simulink model "Versie2"  (R2019a)
settings: Solver=ode1  StartTime=0.0  StopTime=1.5  FixedStep=Ts_Power  RelTol=1e-3
PostLoadFcn:
  | %% Init for wind PnO models - global system parameters
  | OVERRIDE_SSN_MEMORY_LIMIT=1;
  | Ts=50e-6;
  | % Ts=50e-10;
  | Ts_Power=Ts;
  | Ts_Control=2*Ts;
  | freq = 50;
  | Fnom=freq;
  | Vac=400e3;
InitFcn:
  | %% Init for wind PnO models - global system parameters
  | OVERRIDE_SSN_MEMORY_LIMIT=1;
  | Ts=50e-6;
  | % Ts=50e-10;
  | Ts_Power=Ts;
  | Ts_Control=2*Ts;
  | freq = 50;
  | Fnom=freq;
  | Vac=400e3;
undefined symbols (not defined in the file or in its folder): D11, Delta, den, DiscIntNeverNeededParam, dx, find_system, gcbh, num, out_Buses, out_WindFarms, sps_rtmsupport
libraries: powerlib x258, simulink x112, powerlib_meascontrol x112, eeSinusoidalMeasurement x74, spsVIMeasurementModel x63, elements x52, simulink_extras x44, eePowerMeasurement x26
(part 2 of 27)

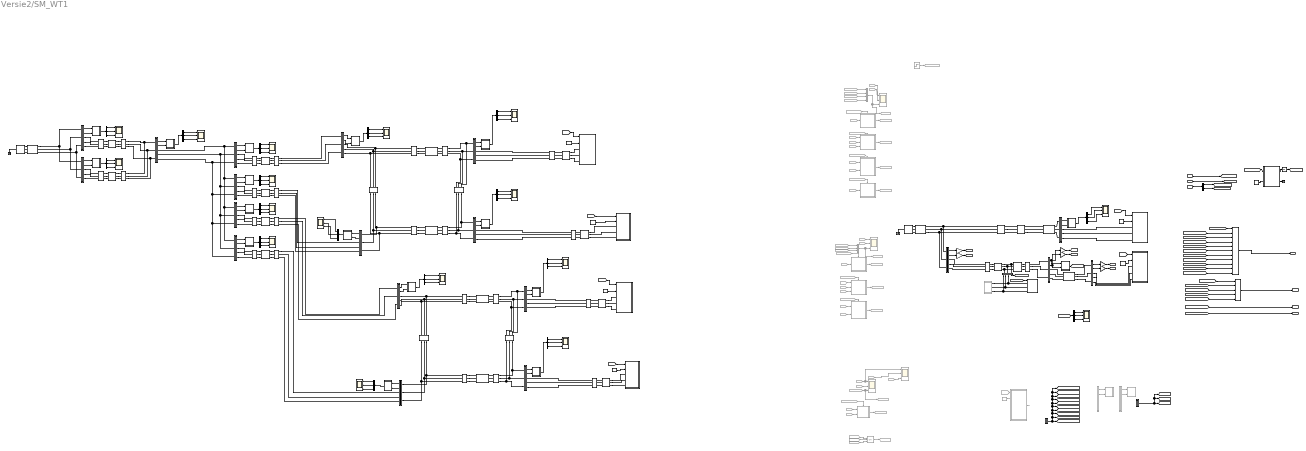
== system Versie2/SM_WT1 ==
  note: Faults
      | with
      | disconnection
      | line
  note: Inputs / Outputs
  note: Analogue Outputs
  note: Digital input (trip signal)
  note: Buses
  note: Wind farms
  note: MODEL TOOLS
  note: Fault
  note: Inputs to this processor core
      | Including blocks to coordinate the communcations
  note: Outputs to monitoring (console)
      | For user interface ('SC_' subsystem)
  note: This subsystem contains the electrical simulation. When performing real-time simulations you cannot view the scopes here. When performing non-real-time simulation (just in matlab/simulink) you can add/view scopes here.
  note: Measurement and protection: bus 2
  note: Measurement and protection: Transformer
  note: Measurement and protection: bus 1
  note: Block protection until model initalised
  wind : Inport
  "FaultParams " : Inport  Port=2
  PlotSelection : Inport  Port=3
   {1..6} (6 alike) : powerlib/Elements/Three-Phase Transformer (Two Windings)  Winding1Connection=Y  Winding2Connection=Yg  CoreType=Three single-phase transformers  SetSaturation=off  Hysteresis=off  DataFile='hysteresis'  SetInitialFlux=off  Measurements=None  UNITS=pu  NominalPower=[1e9 freq]  Winding1=[Vac 0.00083333 0.025]  Winding2=[66e3 0.00083333 0.025]  Rm=500  Lm=Inf  L0=0.5  Saturation=[0 0;0.0024 1.2;1 1.52]  InitialFluxes=[ 0.8 , -0.8 , 0.7 ]  BreakLoop=off  DiscreteSolver=Trapezoidal iterative  DataType=off  TransfoNumber=0
  2500 MVA X0/X1=1 : powerlib/Elements/Three-Phase Mutual Inductance Z1-Z0  LConnTagsString=a|b|c  RConnTagsString=A|B|C  PositiveSequence="[0.1  1.0/(2*pi*freq)] *Vac^2/2500e6/10"  ZeroSequence="[0.3  3.0/(2*pi*freq)] *Vac^2/2500e6/10"
      settings: SourceProductBaseCode=PS
  2500 MVA X0/X1=2 : powerlib/Elements/Three-Phase Mutual Inductance Z1-Z0  LConnTagsString=a|b|c  RConnTagsString=A|B|C  PositiveSequence="[0.1  1.0/(2*pi*freq)] *Vac^2/2500e6/10"  ZeroSequence="[0.3  3.0/(2*pi*freq)] *Vac^2/2500e6/10"
      settings: SourceProductBaseCode=PS
  5 km fault1 : powerlib/Elements/Three-Phase PI Section Line  LConnTagsString=a|b|c  RConnTagsString=A|B|C  Frequency=freq  Resistances=[0.1153 0.413]  Inductances=[1.05e-3 3.32e-3]  Capacitances=[11.33e-009 5.01e-009]  Length=20
  5 km fault2 : powerlib/Elements/Three-Phase PI Section Line  LConnTagsString=a|b|c  RConnTagsString=A|B|C  Frequency=freq  Resistances=[0.1153 0.413]  Inductances=[1.05e-3 3.32e-3]  Capacitances=[11.33e-009 5.01e-009]  Length=20
  5 km series1 : powerlib/Elements/Three-Phase PI Section Line  LConnTagsString=a|b|c  RConnTagsString=A|B|C  Frequency=freq  Resistances=[0.1153 0.413]  Inductances=[1.05e-3 3.32e-3]  Capacitances=[11.33e-009 5.01e-009]  Length=20
  5 km series{3..8,11,17,28,34} (10 alike) : powerlib/Elements/Three-Phase PI Section Line  LConnTagsString=a|b|c  RConnTagsString=A|B|C  Frequency=freq  Resistances=[0.1153 0.413]  Inductances=[1.05e-3 3.32e-3]  Capacitances=[11.33e-009 5.01e-009]  Length=10
  5 km series2 : powerlib/Elements/Three-Phase PI Section Line  LConnTagsString=a|b|c  RConnTagsString=A|B|C  Frequency=freq  Resistances=[0.1153 0.413]  Inductances=[1.05e-3 3.32e-3]  Capacitances=[11.33e-009 5.01e-009]  Length=20
  Bus Creator : BusCreator  Commented=on  Inputs=4
  Bus Creator1 : BusCreator  Commented=on  Inputs=3
  Bus Selector : BusSelector  OutputSignals=Turbine,Bus
  Bus Selector{1..17} (17 alike) : BusSelector  OutputSignals=Vabc,Iabc,PQ
  BusA : Subsystem  DialogController=POWERSYS.PowerSysDialog  LoadFcn=sps_rtmsupport('LoadFcn',gcbh);  StartFcn=sps_rtmsupport('StartFcn',gcbh);  StopFcn=sps_rtmsupport('StopFcn',gcbh);  mask(Three-Phase VI Measurement){VoltageMeasurement=phase-to-ground, SetLabelV=off, LabelV=Vabc, Vpu=off, VpuLL=off, CurrentMeasurement=yes, SetLabelI=off, LabelI=Iabc, Ipu=off, Pbase=100e6, Vbase=500e3, OutputType=Complex, PhasorSimulation=off, PSBequivalent=0}
      mask prompts: VoltageMeasurement "Voltage measurement"; SetLabelV "Use a label"; LabelV "Signal label  (use a From block to collect this signal)"; Vpu "Voltages in pu,  based on peak value of nominal phase-to-ground voltage"; VpuLL "Voltages in pu,  based on peak value of nominal phase-to-phase  voltage"; CurrentMeasurement "Current measurement"; SetLabelI "Use a label"; LabelI "Signal label  (use a From block to collect this signal)"; Ipu "Currents in pu"; Pbase "Base power ( VA 3 phase)"; Vbase "Nominal voltage used for pu measurement (Vrms phase-phase) :"; OutputType "Output signals in:"; PhasorSimulation "Phasor simulation (internal use)"; PSBequivalent "Equivalent circuit (internal use)"
      mask help:
      | Ideal three-phase voltage and current measurements.
      |
      | The block can output the voltages and currents in per unit values or in volts and amperes.
      mask init:
      | block = gcb;
      | Kv=1;
      | Ki=1;
      | [Kv,Ki] = powericon('ThreePhaseVIMeasurementParam',block,Vpu,VpuLL,Ipu,Vbase,Pbase,PhasorSimulation,OutputType);
      | powericon('ThreePhaseVIMeasurementCback',block);
      | power_initmask();
      settings: CopyFcn=sps_rtmsupport('CopyFcn',gcbh); powericon('ThreePhaseVIMeasurementCopy',gcb)  DeleteFcn=sps_rtmsupport('DeleteFcn',gcbh);  UndoDeleteFcn=sps_rtmsupport('UndoDeleteFcn',gcbh);  ModelCloseFcn=sps_rtmsupport('ModelCloseFcn',gcbh);  PreSaveFcn="sps_rtmsupport('PreSaveFcn',gcbh);  set_param(gcb,'LinkStatus','restore')"  PostSaveFcn=sps_rtmsupport('PostSaveFcn',gcbh);  NameChangeFcn=sps_rtmsupport('NameChangeFcn',gcbh);  PreCopyFcn=sps_rtmsupport('PreCopyFcn',gcbh);  OpenFcn=sps_rtmsupport('OpenFcn',gcbh, [1 2 4 5 6 7 9 -12 13]);  CloseFcn=sps_rtmsupport('CloseFcn',gcbh);  PreDeleteFcn=sps_rtmsupport('PreDeleteFcn',gcbh);
      mask Help: helpview(psbhelp)
      mask TypeOptions VoltageMeasurement: no | phase-to-ground | phase-to-phase
      mask Callback VoltageMeasurement: powericon('ThreePhaseVIMeasurementCback',gcb,'Vselector');
      mask Callback SetLabelV: powericon('ThreePhaseVIMeasurementCback',gcb,'');
      mask Callback Vpu: powericon('ThreePhaseVIMeasurementCback',gcb,'Vpu');
      mask Callback VpuLL: powericon('ThreePhaseVIMeasurementCback',gcb,'VpuLL');
      mask TypeOptions CurrentMeasurement: no | yes
      mask Callback CurrentMeasurement: powericon('ThreePhaseVIMeasurementCback',gcb,'');
      mask Callback SetLabelI: powericon('ThreePhaseVIMeasurementCback',gcb,'');
      mask Callback LabelI: powericon('ThreePhaseVIMeasurementCback',gcb,'');
      mask Callback Ipu: powericon('ThreePhaseVIMeasurementCback',gcb,'');
      mask TypeOptions OutputType: Complex | Real-Imag | Magnitude-Angle | Magnitude
  BusB : Subsystem  Commented=on  DialogController=POWERSYS.PowerSysDialog  LoadFcn=sps_rtmsupport('LoadFcn',gcbh);  StartFcn=sps_rtmsupport('StartFcn',gcbh);  StopFcn=sps_rtmsupport('StopFcn',gcbh);  mask(Three-Phase VI Measurement){VoltageMeasurement=phase-to-ground, SetLabelV=off, LabelV=Vabc, Vpu=off, VpuLL=off, CurrentMeasurement=yes, SetLabelI=off, LabelI=Iabc, Ipu=off, Pbase=100e6, Vbase=500e3, OutputType=Complex, PhasorSimulation=off, PSBequivalent=0}
      mask prompts: VoltageMeasurement "Voltage measurement"; SetLabelV "Use a label"; LabelV "Signal label  (use a From block to collect this signal)"; Vpu "Voltages in pu,  based on peak value of nominal phase-to-ground voltage"; VpuLL "Voltages in pu,  based on peak value of nominal phase-to-phase  voltage"; CurrentMeasurement "Current measurement"; SetLabelI "Use a label"; LabelI "Signal label  (use a From block to collect this signal)"; Ipu "Currents in pu"; Pbase "Base power ( VA 3 phase)"; Vbase "Nominal voltage used for pu measurement (Vrms phase-phase) :"; OutputType "Output signals in:"; PhasorSimulation "Phasor simulation (internal use)"; PSBequivalent "Equivalent circuit (internal use)"
      mask help:
      | Ideal three-phase voltage and current measurements.
      |
      | The block can output the voltages and currents in per unit values or in volts and amperes.
      mask init: same as Versie2/SM_WT1/BusA
      settings: CopyFcn=sps_rtmsupport('CopyFcn',gcbh); powericon('ThreePhaseVIMeasurementCopy',gcb)  DeleteFcn=sps_rtmsupport('DeleteFcn',gcbh);  UndoDeleteFcn=sps_rtmsupport('UndoDeleteFcn',gcbh);  ModelCloseFcn=sps_rtmsupport('ModelCloseFcn',gcbh);  PreSaveFcn="sps_rtmsupport('PreSaveFcn',gcbh);  set_param(gcb,'LinkStatus','restore')"  PostSaveFcn=sps_rtmsupport('PostSaveFcn',gcbh);  NameChangeFcn=sps_rtmsupport('NameChangeFcn',gcbh);  PreCopyFcn=sps_rtmsupport('PreCopyFcn',gcbh);  OpenFcn=sps_rtmsupport('OpenFcn',gcbh, [1 2 4 5 6 7 9 -12 13]);  CloseFcn=sps_rtmsupport('CloseFcn',gcbh);  PreDeleteFcn=sps_rtmsupport('PreDeleteFcn',gcbh);
      mask Help: helpview(psbhelp)
      mask TypeOptions VoltageMeasurement: no | phase-to-ground | phase-to-phase
      mask Callback VoltageMeasurement: powericon('ThreePhaseVIMeasurementCback',gcb,'Vselector');
      mask Callback SetLabelV: powericon('ThreePhaseVIMeasurementCback',gcb,'');
      mask Callback Vpu: powericon('ThreePhaseVIMeasurementCback',gcb,'Vpu');
      mask Callback VpuLL: powericon('ThreePhaseVIMeasurementCback',gcb,'VpuLL');
      mask TypeOptions CurrentMeasurement: no | yes
      mask Callback CurrentMeasurement: powericon('ThreePhaseVIMeasurementCback',gcb,'');
      mask Callback SetLabelI: powericon('ThreePhaseVIMeasurementCback',gcb,'');
      mask Callback LabelI: powericon('ThreePhaseVIMeasurementCback',gcb,'');
      mask Callback Ipu: powericon('ThreePhaseVIMeasurementCback',gcb,'');
      mask TypeOptions OutputType: Complex | Real-Imag | Magnitude-Angle | Magnitude
  BusC : Subsystem  DialogController=POWERSYS.PowerSysDialog  LoadFcn=sps_rtmsupport('LoadFcn',gcbh);  StartFcn=sps_rtmsupport('StartFcn',gcbh);  StopFcn=sps_rtmsupport('StopFcn',gcbh);  mask(Three-Phase VI Measurement){VoltageMeasurement=phase-to-ground, SetLabelV=off, LabelV=Vabc, Vpu=off, VpuLL=off, CurrentMeasurement=yes, SetLabelI=off, LabelI=Iabc, Ipu=off, Pbase=100e6, Vbase=500e3, OutputType=Complex, PhasorSimulation=off, PSBequivalent=0}
      mask prompts: VoltageMeasurement "Voltage measurement"; SetLabelV "Use a label"; LabelV "Signal label  (use a From block to collect this signal)"; Vpu "Voltages in pu,  based on peak value of nominal phase-to-ground voltage"; VpuLL "Voltages in pu,  based on peak value of nominal phase-to-phase  voltage"; CurrentMeasurement "Current measurement"; SetLabelI "Use a label"; LabelI "Signal label  (use a From block to collect this signal)"; Ipu "Currents in pu"; Pbase "Base power ( VA 3 phase)"; Vbase "Nominal voltage used for pu measurement (Vrms phase-phase) :"; OutputType "Output signals in:"; PhasorSimulation "Phasor simulation (internal use)"; PSBequivalent "Equivalent circuit (internal use)"
      mask help:
      | Ideal three-phase voltage and current measurements.
      |
      | The block can output the voltages and currents in per unit values or in volts and amperes.
      mask init: same as Versie2/SM_WT1/BusA
      settings: CopyFcn=sps_rtmsupport('CopyFcn',gcbh); powericon('ThreePhaseVIMeasurementCopy',gcb)  DeleteFcn=sps_rtmsupport('DeleteFcn',gcbh);  UndoDeleteFcn=sps_rtmsupport('UndoDeleteFcn',gcbh);  ModelCloseFcn=sps_rtmsupport('ModelCloseFcn',gcbh);  PreSaveFcn="sps_rtmsupport('PreSaveFcn',gcbh);  set_param(gcb,'LinkStatus','restore')"  PostSaveFcn=sps_rtmsupport('PostSaveFcn',gcbh);  NameChangeFcn=sps_rtmsupport('NameChangeFcn',gcbh);  PreCopyFcn=sps_rtmsupport('PreCopyFcn',gcbh);  OpenFcn=sps_rtmsupport('OpenFcn',gcbh, [1 2 4 5 6 7 9 -12 13]);  CloseFcn=sps_rtmsupport('CloseFcn',gcbh);  PreDeleteFcn=sps_rtmsupport('PreDeleteFcn',gcbh);
      mask Help: helpview(psbhelp)
      mask TypeOptions VoltageMeasurement: no | phase-to-ground | phase-to-phase
      mask Callback VoltageMeasurement: powericon('ThreePhaseVIMeasurementCback',gcb,'Vselector');
      mask Callback SetLabelV: powericon('ThreePhaseVIMeasurementCback',gcb,'');
      mask Callback Vpu: powericon('ThreePhaseVIMeasurementCback',gcb,'Vpu');
      mask Callback VpuLL: powericon('ThreePhaseVIMeasurementCback',gcb,'VpuLL');
      mask TypeOptions CurrentMeasurement: no | yes
      mask Callback CurrentMeasurement: powericon('ThreePhaseVIMeasurementCback',gcb,'');
      mask Callback SetLabelI: powericon('ThreePhaseVIMeasurementCback',gcb,'');
      mask Callback LabelI: powericon('ThreePhaseVIMeasurementCback',gcb,'');
      mask Callback Ipu: powericon('ThreePhaseVIMeasurementCback',gcb,'');
      mask TypeOptions OutputType: Complex | Real-Imag | Magnitude-Angle | Magnitude
  BusC1 : Subsystem  DialogController=POWERSYS.PowerSysDialog  LoadFcn=sps_rtmsupport('LoadFcn',gcbh);  StartFcn=sps_rtmsupport('StartFcn',gcbh);  StopFcn=sps_rtmsupport('StopFcn',gcbh);  mask(Three-Phase VI Measurement){VoltageMeasurement=phase-to-ground, SetLabelV=off, LabelV=Vabc, Vpu=off, VpuLL=off, CurrentMeasurement=yes, SetLabelI=off, LabelI=Iabc, Ipu=off, Pbase=100e6, Vbase=500e3, OutputType=Complex, PhasorSimulation=off, PSBequivalent=0}
      mask prompts: VoltageMeasurement "Voltage measurement"; SetLabelV "Use a label"; LabelV "Signal label  (use a From block to collect this signal)"; Vpu "Voltages in pu,  based on peak value of nominal phase-to-ground voltage"; VpuLL "Voltages in pu,  based on peak value of nominal phase-to-phase  voltage"; CurrentMeasurement "Current measurement"; SetLabelI "Use a label"; LabelI "Signal label  (use a From block to collect this signal)"; Ipu "Currents in pu"; Pbase "Base power ( VA 3 phase)"; Vbase "Nominal voltage used for pu measurement (Vrms phase-phase) :"; OutputType "Output signals in:"; PhasorSimulation "Phasor simulation (internal use)"; PSBequivalent "Equivalent circuit (internal use)"
      mask help:
      | Ideal three-phase voltage and current measurements.
      |
      | The block can output the voltages and currents in per unit values or in volts and amperes.
      mask init: same as Versie2/SM_WT1/BusA
      settings: CopyFcn=sps_rtmsupport('CopyFcn',gcbh); powericon('ThreePhaseVIMeasurementCopy',gcb)  DeleteFcn=sps_rtmsupport('DeleteFcn',gcbh);  UndoDeleteFcn=sps_rtmsupport('UndoDeleteFcn',gcbh);  ModelCloseFcn=sps_rtmsupport('ModelCloseFcn',gcbh);  PreSaveFcn="sps_rtmsupport('PreSaveFcn',gcbh);  set_param(gcb,'LinkStatus','restore')"  PostSaveFcn=sps_rtmsupport('PostSaveFcn',gcbh);  NameChangeFcn=sps_rtmsupport('NameChangeFcn',gcbh);  PreCopyFcn=sps_rtmsupport('PreCopyFcn',gcbh);  OpenFcn=sps_rtmsupport('OpenFcn',gcbh, [1 2 4 5 6 7 9 -12 13]);  CloseFcn=sps_rtmsupport('CloseFcn',gcbh);  PreDeleteFcn=sps_rtmsupport('PreDeleteFcn',gcbh);
      mask Help: helpview(psbhelp)
      mask TypeOptions VoltageMeasurement: no | phase-to-ground | phase-to-phase
      mask Callback VoltageMeasurement: powericon('ThreePhaseVIMeasurementCback',gcb,'Vselector');
      mask Callback SetLabelV: powericon('ThreePhaseVIMeasurementCback',gcb,'');
      mask Callback Vpu: powericon('ThreePhaseVIMeasurementCback',gcb,'Vpu');
      mask Callback VpuLL: powericon('ThreePhaseVIMeasurementCback',gcb,'VpuLL');
      mask TypeOptions CurrentMeasurement: no | yes
      mask Callback CurrentMeasurement: powericon('ThreePhaseVIMeasurementCback',gcb,'');
      mask Callback SetLabelI: powericon('ThreePhaseVIMeasurementCback',gcb,'');
      mask Callback LabelI: powericon('ThreePhaseVIMeasurementCback',gcb,'');
      mask Callback Ipu: powericon('ThreePhaseVIMeasurementCback',gcb,'');
      mask TypeOptions OutputType: Complex | Real-Imag | Magnitude-Angle | Magnitude
  BusC10 : Subsystem  DialogController=POWERSYS.PowerSysDialog  LoadFcn=sps_rtmsupport('LoadFcn',gcbh);  StartFcn=sps_rtmsupport('StartFcn',gcbh);  StopFcn=sps_rtmsupport('StopFcn',gcbh);  mask(Three-Phase VI Measurement){VoltageMeasurement=phase-to-ground, SetLabelV=off, LabelV=Vabc, Vpu=off, VpuLL=off, CurrentMeasurement=yes, SetLabelI=off, LabelI=Iabc, Ipu=off, Pbase=100e6, Vbase=500e3, OutputType=Complex, PhasorSimulation=off, PSBequivalent=0}
      mask prompts: VoltageMeasurement "Voltage measurement"; SetLabelV "Use a label"; LabelV "Signal label  (use a From block to collect this signal)"; Vpu "Voltages in pu,  based on peak value of nominal phase-to-ground voltage"; VpuLL "Voltages in pu,  based on peak value of nominal phase-to-phase  voltage"; CurrentMeasurement "Current measurement"; SetLabelI "Use a label"; LabelI "Signal label  (use a From block to collect this signal)"; Ipu "Currents in pu"; Pbase "Base power ( VA 3 phase)"; Vbase "Nominal voltage used for pu measurement (Vrms phase-phase) :"; OutputType "Output signals in:"; PhasorSimulation "Phasor simulation (internal use)"; PSBequivalent "Equivalent circuit (internal use)"
      mask help:
      | Ideal three-phase voltage and current measurements.
      |
      | The block can output the voltages and currents in per unit values or in volts and amperes.
      mask init: same as Versie2/SM_WT1/BusA
      settings: CopyFcn=sps_rtmsupport('CopyFcn',gcbh); powericon('ThreePhaseVIMeasurementCopy',gcb)  DeleteFcn=sps_rtmsupport('DeleteFcn',gcbh);  UndoDeleteFcn=sps_rtmsupport('UndoDeleteFcn',gcbh);  ModelCloseFcn=sps_rtmsupport('ModelCloseFcn',gcbh);  PreSaveFcn="sps_rtmsupport('PreSaveFcn',gcbh);  set_param(gcb,'LinkStatus','restore')"  PostSaveFcn=sps_rtmsupport('PostSaveFcn',gcbh);  NameChangeFcn=sps_rtmsupport('NameChangeFcn',gcbh);  PreCopyFcn=sps_rtmsupport('PreCopyFcn',gcbh);  OpenFcn=sps_rtmsupport('OpenFcn',gcbh, [1 2 4 5 6 7 9 -12 13]);  CloseFcn=sps_rtmsupport('CloseFcn',gcbh);  PreDeleteFcn=sps_rtmsupport('PreDeleteFcn',gcbh);
      mask Help: helpview(psbhelp)
      mask TypeOptions VoltageMeasurement: no | phase-to-ground | phase-to-phase
      mask Callback VoltageMeasurement: powericon('ThreePhaseVIMeasurementCback',gcb,'Vselector');
      mask Callback SetLabelV: powericon('ThreePhaseVIMeasurementCback',gcb,'');
      mask Callback Vpu: powericon('ThreePhaseVIMeasurementCback',gcb,'Vpu');
      mask Callback VpuLL: powericon('ThreePhaseVIMeasurementCback',gcb,'VpuLL');
      mask TypeOptions CurrentMeasurement: no | yes
      mask Callback CurrentMeasurement: powericon('ThreePhaseVIMeasurementCback',gcb,'');
      mask Callback SetLabelI: powericon('ThreePhaseVIMeasurementCback',gcb,'');
      mask Callback LabelI: powericon('ThreePhaseVIMeasurementCback',gcb,'');
      mask Callback Ipu: powericon('ThreePhaseVIMeasurementCback',gcb,'');
      mask TypeOptions OutputType: Complex | Real-Imag | Magnitude-Angle | Magnitude
  BusC11 : Subsystem  DialogController=POWERSYS.PowerSysDialog  LoadFcn=sps_rtmsupport('LoadFcn',gcbh);  StartFcn=sps_rtmsupport('StartFcn',gcbh);  StopFcn=sps_rtmsupport('StopFcn',gcbh);  mask(Three-Phase VI Measurement){VoltageMeasurement=phase-to-ground, SetLabelV=off, LabelV=Vabc, Vpu=off, VpuLL=off, CurrentMeasurement=yes, SetLabelI=off, LabelI=Iabc, Ipu=off, Pbase=100e6, Vbase=500e3, OutputType=Complex, PhasorSimulation=off, PSBequivalent=0}
      mask prompts: VoltageMeasurement "Voltage measurement"; SetLabelV "Use a label"; LabelV "Signal label  (use a From block to collect this signal)"; Vpu "Voltages in pu,  based on peak value of nominal phase-to-ground voltage"; VpuLL "Voltages in pu,  based on peak value of nominal phase-to-phase  voltage"; CurrentMeasurement "Current measurement"; SetLabelI "Use a label"; LabelI "Signal label  (use a From block to collect this signal)"; Ipu "Currents in pu"; Pbase "Base power ( VA 3 phase)"; Vbase "Nominal voltage used for pu measurement (Vrms phase-phase) :"; OutputType "Output signals in:"; PhasorSimulation "Phasor simulation (internal use)"; PSBequivalent "Equivalent circuit (internal use)"
      mask help:
      | Ideal three-phase voltage and current measurements.
      |
      | The block can output the voltages and currents in per unit values or in volts and amperes.
      mask init: same as Versie2/SM_WT1/BusA
      settings: CopyFcn=sps_rtmsupport('CopyFcn',gcbh); powericon('ThreePhaseVIMeasurementCopy',gcb)  DeleteFcn=sps_rtmsupport('DeleteFcn',gcbh);  UndoDeleteFcn=sps_rtmsupport('UndoDeleteFcn',gcbh);  ModelCloseFcn=sps_rtmsupport('ModelCloseFcn',gcbh);  PreSaveFcn="sps_rtmsupport('PreSaveFcn',gcbh);  set_param(gcb,'LinkStatus','restore')"  PostSaveFcn=sps_rtmsupport('PostSaveFcn',gcbh);  NameChangeFcn=sps_rtmsupport('NameChangeFcn',gcbh);  PreCopyFcn=sps_rtmsupport('PreCopyFcn',gcbh);  OpenFcn=sps_rtmsupport('OpenFcn',gcbh, [1 2 4 5 6 7 9 -12 13]);  CloseFcn=sps_rtmsupport('CloseFcn',gcbh);  PreDeleteFcn=sps_rtmsupport('PreDeleteFcn',gcbh);
      mask Help: helpview(psbhelp)
      mask TypeOptions VoltageMeasurement: no | phase-to-ground | phase-to-phase
      mask Callback VoltageMeasurement: powericon('ThreePhaseVIMeasurementCback',gcb,'Vselector');
      mask Callback SetLabelV: powericon('ThreePhaseVIMeasurementCback',gcb,'');
      mask Callback Vpu: powericon('ThreePhaseVIMeasurementCback',gcb,'Vpu');
      mask Callback VpuLL: powericon('ThreePhaseVIMeasurementCback',gcb,'VpuLL');
      mask TypeOptions CurrentMeasurement: no | yes
      mask Callback CurrentMeasurement: powericon('ThreePhaseVIMeasurementCback',gcb,'');
      mask Callback SetLabelI: powericon('ThreePhaseVIMeasurementCback',gcb,'');
      mask Callback LabelI: powericon('ThreePhaseVIMeasurementCback',gcb,'');
      mask Callback Ipu: powericon('ThreePhaseVIMeasurementCback',gcb,'');
      mask TypeOptions OutputType: Complex | Real-Imag | Magnitude-Angle | Magnitude
  BusC12 : Subsystem  DialogController=POWERSYS.PowerSysDialog  LoadFcn=sps_rtmsupport('LoadFcn',gcbh);  StartFcn=sps_rtmsupport('StartFcn',gcbh);  StopFcn=sps_rtmsupport('StopFcn',gcbh);  mask(Three-Phase VI Measurement){VoltageMeasurement=phase-to-ground, SetLabelV=off, LabelV=Vabc, Vpu=off, VpuLL=off, CurrentMeasurement=yes, SetLabelI=off, LabelI=Iabc, Ipu=off, Pbase=100e6, Vbase=500e3, OutputType=Complex, PhasorSimulation=off, PSBequivalent=0}
      mask prompts: VoltageMeasurement "Voltage measurement"; SetLabelV "Use a label"; LabelV "Signal label  (use a From block to collect this signal)"; Vpu "Voltages in pu,  based on peak value of nominal phase-to-ground voltage"; VpuLL "Voltages in pu,  based on peak value of nominal phase-to-phase  voltage"; CurrentMeasurement "Current measurement"; SetLabelI "Use a label"; LabelI "Signal label  (use a From block to collect this signal)"; Ipu "Currents in pu"; Pbase "Base power ( VA 3 phase)"; Vbase "Nominal voltage used for pu measurement (Vrms phase-phase) :"; OutputType "Output signals in:"; PhasorSimulation "Phasor simulation (internal use)"; PSBequivalent "Equivalent circuit (internal use)"
      mask help:
      | Ideal three-phase voltage and current measurements.
      |
      | The block can output the voltages and currents in per unit values or in volts and amperes.
      mask init: same as Versie2/SM_WT1/BusA
      settings: CopyFcn=sps_rtmsupport('CopyFcn',gcbh); powericon('ThreePhaseVIMeasurementCopy',gcb)  DeleteFcn=sps_rtmsupport('DeleteFcn',gcbh);  UndoDeleteFcn=sps_rtmsupport('UndoDeleteFcn',gcbh);  ModelCloseFcn=sps_rtmsupport('ModelCloseFcn',gcbh);  PreSaveFcn="sps_rtmsupport('PreSaveFcn',gcbh);  set_param(gcb,'LinkStatus','restore')"  PostSaveFcn=sps_rtmsupport('PostSaveFcn',gcbh);  NameChangeFcn=sps_rtmsupport('NameChangeFcn',gcbh);  PreCopyFcn=sps_rtmsupport('PreCopyFcn',gcbh);  OpenFcn=sps_rtmsupport('OpenFcn',gcbh, [1 2 4 5 6 7 9 -12 13]);  CloseFcn=sps_rtmsupport('CloseFcn',gcbh);  PreDeleteFcn=sps_rtmsupport('PreDeleteFcn',gcbh);
      mask Help: helpview(psbhelp)
      mask TypeOptions VoltageMeasurement: no | phase-to-ground | phase-to-phase
      mask Callback VoltageMeasurement: powericon('ThreePhaseVIMeasurementCback',gcb,'Vselector');
      mask Callback SetLabelV: powericon('ThreePhaseVIMeasurementCback',gcb,'');
      mask Callback Vpu: powericon('ThreePhaseVIMeasurementCback',gcb,'Vpu');
      mask Callback VpuLL: powericon('ThreePhaseVIMeasurementCback',gcb,'VpuLL');
      mask TypeOptions CurrentMeasurement: no | yes
      mask Callback CurrentMeasurement: powericon('ThreePhaseVIMeasurementCback',gcb,'');
      mask Callback SetLabelI: powericon('ThreePhaseVIMeasurementCback',gcb,'');
      mask Callback LabelI: powericon('ThreePhaseVIMeasurementCback',gcb,'');
      mask Callback Ipu: powericon('ThreePhaseVIMeasurementCback',gcb,'');
      mask TypeOptions OutputType: Complex | Real-Imag | Magnitude-Angle | Magnitude
  BusC13 : Subsystem  DialogController=POWERSYS.PowerSysDialog  LoadFcn=sps_rtmsupport('LoadFcn',gcbh);  StartFcn=sps_rtmsupport('StartFcn',gcbh);  StopFcn=sps_rtmsupport('StopFcn',gcbh);  mask(Three-Phase VI Measurement){VoltageMeasurement=phase-to-ground, SetLabelV=off, LabelV=Vabc, Vpu=off, VpuLL=off, CurrentMeasurement=yes, SetLabelI=off, LabelI=Iabc, Ipu=off, Pbase=100e6, Vbase=500e3, OutputType=Complex, PhasorSimulation=off, PSBequivalent=0}
      mask prompts: VoltageMeasurement "Voltage measurement"; SetLabelV "Use a label"; LabelV "Signal label  (use a From block to collect this signal)"; Vpu "Voltages in pu,  based on peak value of nominal phase-to-ground voltage"; VpuLL "Voltages in pu,  based on peak value of nominal phase-to-phase  voltage"; CurrentMeasurement "Current measurement"; SetLabelI "Use a label"; LabelI "Signal label  (use a From block to collect this signal)"; Ipu "Currents in pu"; Pbase "Base power ( VA 3 phase)"; Vbase "Nominal voltage used for pu measurement (Vrms phase-phase) :"; OutputType "Output signals in:"; PhasorSimulation "Phasor simulation (internal use)"; PSBequivalent "Equivalent circuit (internal use)"
      mask help:
      | Ideal three-phase voltage and current measurements.
      |
      | The block can output the voltages and currents in per unit values or in volts and amperes.
      mask init: same as Versie2/SM_WT1/BusA
      settings: CopyFcn=sps_rtmsupport('CopyFcn',gcbh); powericon('ThreePhaseVIMeasurementCopy',gcb)  DeleteFcn=sps_rtmsupport('DeleteFcn',gcbh);  UndoDeleteFcn=sps_rtmsupport('UndoDeleteFcn',gcbh);  ModelCloseFcn=sps_rtmsupport('ModelCloseFcn',gcbh);  PreSaveFcn="sps_rtmsupport('PreSaveFcn',gcbh);  set_param(gcb,'LinkStatus','restore')"  PostSaveFcn=sps_rtmsupport('PostSaveFcn',gcbh);  NameChangeFcn=sps_rtmsupport('NameChangeFcn',gcbh);  PreCopyFcn=sps_rtmsupport('PreCopyFcn',gcbh);  OpenFcn=sps_rtmsupport('OpenFcn',gcbh, [1 2 4 5 6 7 9 -12 13]);  CloseFcn=sps_rtmsupport('CloseFcn',gcbh);  PreDeleteFcn=sps_rtmsupport('PreDeleteFcn',gcbh);
      mask Help: helpview(psbhelp)
      mask TypeOptions VoltageMeasurement: no | phase-to-ground | phase-to-phase
      mask Callback VoltageMeasurement: powericon('ThreePhaseVIMeasurementCback',gcb,'Vselector');
      mask Callback SetLabelV: powericon('ThreePhaseVIMeasurementCback',gcb,'');
      mask Callback Vpu: powericon('ThreePhaseVIMeasurementCback',gcb,'Vpu');
      mask Callback VpuLL: powericon('ThreePhaseVIMeasurementCback',gcb,'VpuLL');
      mask TypeOptions CurrentMeasurement: no | yes
      mask Callback CurrentMeasurement: powericon('ThreePhaseVIMeasurementCback',gcb,'');
      mask Callback SetLabelI: powericon('ThreePhaseVIMeasurementCback',gcb,'');
      mask Callback LabelI: powericon('ThreePhaseVIMeasurementCback',gcb,'');
      mask Callback Ipu: powericon('ThreePhaseVIMeasurementCback',gcb,'');
      mask TypeOptions OutputType: Complex | Real-Imag | Magnitude-Angle | Magnitude
  BusC14 : Subsystem  DialogController=POWERSYS.PowerSysDialog  LoadFcn=sps_rtmsupport('LoadFcn',gcbh);  StartFcn=sps_rtmsupport('StartFcn',gcbh);  StopFcn=sps_rtmsupport('StopFcn',gcbh);  mask(Three-Phase VI Measurement){VoltageMeasurement=phase-to-ground, SetLabelV=off, LabelV=Vabc, Vpu=off, VpuLL=off, CurrentMeasurement=yes, SetLabelI=off, LabelI=Iabc, Ipu=off, Pbase=100e6, Vbase=500e3, OutputType=Complex, PhasorSimulation=off, PSBequivalent=0}
      mask prompts: VoltageMeasurement "Voltage measurement"; SetLabelV "Use a label"; LabelV "Signal label  (use a From block to collect this signal)"; Vpu "Voltages in pu,  based on peak value of nominal phase-to-ground voltage"; VpuLL "Voltages in pu,  based on peak value of nominal phase-to-phase  voltage"; CurrentMeasurement "Current measurement"; SetLabelI "Use a label"; LabelI "Signal label  (use a From block to collect this signal)"; Ipu "Currents in pu"; Pbase "Base power ( VA 3 phase)"; Vbase "Nominal voltage used for pu measurement (Vrms phase-phase) :"; OutputType "Output signals in:"; PhasorSimulation "Phasor simulation (internal use)"; PSBequivalent "Equivalent circuit (internal use)"
      mask help:
      | Ideal three-phase voltage and current measurements.
      |
      | The block can output the voltages and currents in per unit values or in volts and amperes.
      mask init: same as Versie2/SM_WT1/BusA
      settings: CopyFcn=sps_rtmsupport('CopyFcn',gcbh); powericon('ThreePhaseVIMeasurementCopy',gcb)  DeleteFcn=sps_rtmsupport('DeleteFcn',gcbh);  UndoDeleteFcn=sps_rtmsupport('UndoDeleteFcn',gcbh);  ModelCloseFcn=sps_rtmsupport('ModelCloseFcn',gcbh);  PreSaveFcn="sps_rtmsupport('PreSaveFcn',gcbh);  set_param(gcb,'LinkStatus','restore')"  PostSaveFcn=sps_rtmsupport('PostSaveFcn',gcbh);  NameChangeFcn=sps_rtmsupport('NameChangeFcn',gcbh);  PreCopyFcn=sps_rtmsupport('PreCopyFcn',gcbh);  OpenFcn=sps_rtmsupport('OpenFcn',gcbh, [1 2 4 5 6 7 9 -12 13]);  CloseFcn=sps_rtmsupport('CloseFcn',gcbh);  PreDeleteFcn=sps_rtmsupport('PreDeleteFcn',gcbh);
      mask Help: helpview(psbhelp)
      mask TypeOptions VoltageMeasurement: no | phase-to-ground | phase-to-phase
      mask Callback VoltageMeasurement: powericon('ThreePhaseVIMeasurementCback',gcb,'Vselector');
      mask Callback SetLabelV: powericon('ThreePhaseVIMeasurementCback',gcb,'');
      mask Callback Vpu: powericon('ThreePhaseVIMeasurementCback',gcb,'Vpu');
      mask Callback VpuLL: powericon('ThreePhaseVIMeasurementCback',gcb,'VpuLL');
      mask TypeOptions CurrentMeasurement: no | yes
      mask Callback CurrentMeasurement: powericon('ThreePhaseVIMeasurementCback',gcb,'');
      mask Callback SetLabelI: powericon('ThreePhaseVIMeasurementCback',gcb,'');
      mask Callback LabelI: powericon('ThreePhaseVIMeasurementCback',gcb,'');
      mask Callback Ipu: powericon('ThreePhaseVIMeasurementCback',gcb,'');
      mask TypeOptions OutputType: Complex | Real-Imag | Magnitude-Angle | Magnitude
  BusC15 : Subsystem  DialogController=POWERSYS.PowerSysDialog  LoadFcn=sps_rtmsupport('LoadFcn',gcbh);  StartFcn=sps_rtmsupport('StartFcn',gcbh);  StopFcn=sps_rtmsupport('StopFcn',gcbh);  mask(Three-Phase VI Measurement){VoltageMeasurement=phase-to-ground, SetLabelV=off, LabelV=Vabc, Vpu=off, VpuLL=off, CurrentMeasurement=yes, SetLabelI=off, LabelI=Iabc, Ipu=off, Pbase=100e6, Vbase=500e3, OutputType=Complex, PhasorSimulation=off, PSBequivalent=0}
      mask prompts: VoltageMeasurement "Voltage measurement"; SetLabelV "Use a label"; LabelV "Signal label  (use a From block to collect this signal)"; Vpu "Voltages in pu,  based on peak value of nominal phase-to-ground voltage"; VpuLL "Voltages in pu,  based on peak value of nominal phase-to-phase  voltage"; CurrentMeasurement "Current measurement"; SetLabelI "Use a label"; LabelI "Signal label  (use a From block to collect this signal)"; Ipu "Currents in pu"; Pbase "Base power ( VA 3 phase)"; Vbase "Nominal voltage used for pu measurement (Vrms phase-phase) :"; OutputType "Output signals in:"; PhasorSimulation "Phasor simulation (internal use)"; PSBequivalent "Equivalent circuit (internal use)"
      mask help:
      | Ideal three-phase voltage and current measurements.
      |
      | The block can output the voltages and currents in per unit values or in volts and amperes.
      mask init: same as Versie2/SM_WT1/BusA
      settings: CopyFcn=sps_rtmsupport('CopyFcn',gcbh); powericon('ThreePhaseVIMeasurementCopy',gcb)  DeleteFcn=sps_rtmsupport('DeleteFcn',gcbh);  UndoDeleteFcn=sps_rtmsupport('UndoDeleteFcn',gcbh);  ModelCloseFcn=sps_rtmsupport('ModelCloseFcn',gcbh);  PreSaveFcn="sps_rtmsupport('PreSaveFcn',gcbh);  set_param(gcb,'LinkStatus','restore')"  PostSaveFcn=sps_rtmsupport('PostSaveFcn',gcbh);  NameChangeFcn=sps_rtmsupport('NameChangeFcn',gcbh);  PreCopyFcn=sps_rtmsupport('PreCopyFcn',gcbh);  OpenFcn=sps_rtmsupport('OpenFcn',gcbh, [1 2 4 5 6 7 9 -12 13]);  CloseFcn=sps_rtmsupport('CloseFcn',gcbh);  PreDeleteFcn=sps_rtmsupport('PreDeleteFcn',gcbh);
      mask Help: helpview(psbhelp)
      mask TypeOptions VoltageMeasurement: no | phase-to-ground | phase-to-phase
      mask Callback VoltageMeasurement: powericon('ThreePhaseVIMeasurementCback',gcb,'Vselector');
      mask Callback SetLabelV: powericon('ThreePhaseVIMeasurementCback',gcb,'');
      mask Callback Vpu: powericon('ThreePhaseVIMeasurementCback',gcb,'Vpu');
      mask Callback VpuLL: powericon('ThreePhaseVIMeasurementCback',gcb,'VpuLL');
      mask TypeOptions CurrentMeasurement: no | yes
      mask Callback CurrentMeasurement: powericon('ThreePhaseVIMeasurementCback',gcb,'');
      mask Callback SetLabelI: powericon('ThreePhaseVIMeasurementCback',gcb,'');
      mask Callback LabelI: powericon('ThreePhaseVIMeasurementCback',gcb,'');
      mask Callback Ipu: powericon('ThreePhaseVIMeasurementCback',gcb,'');
      mask TypeOptions OutputType: Complex | Real-Imag | Magnitude-Angle | Magnitude
  BusC16 : Subsystem  DialogController=POWERSYS.PowerSysDialog  LoadFcn=sps_rtmsupport('LoadFcn',gcbh);  StartFcn=sps_rtmsupport('StartFcn',gcbh);  StopFcn=sps_rtmsupport('StopFcn',gcbh);  mask(Three-Phase VI Measurement){VoltageMeasurement=phase-to-ground, SetLabelV=off, LabelV=Vabc, Vpu=off, VpuLL=off, CurrentMeasurement=yes, SetLabelI=off, LabelI=Iabc, Ipu=off, Pbase=100e6, Vbase=500e3, OutputType=Complex, PhasorSimulation=off, PSBequivalent=0}
      mask prompts: VoltageMeasurement "Voltage measurement"; SetLabelV "Use a label"; LabelV "Signal label  (use a From block to collect this signal)"; Vpu "Voltages in pu,  based on peak value of nominal phase-to-ground voltage"; VpuLL "Voltages in pu,  based on peak value of nominal phase-to-phase  voltage"; CurrentMeasurement "Current measurement"; SetLabelI "Use a label"; LabelI "Signal label  (use a From block to collect this signal)"; Ipu "Currents in pu"; Pbase "Base power ( VA 3 phase)"; Vbase "Nominal voltage used for pu measurement (Vrms phase-phase) :"; OutputType "Output signals in:"; PhasorSimulation "Phasor simulation (internal use)"; PSBequivalent "Equivalent circuit (internal use)"
      mask help:
      | Ideal three-phase voltage and current measurements.
      |
      | The block can output the voltages and currents in per unit values or in volts and amperes.
      mask init: same as Versie2/SM_WT1/BusA
      settings: CopyFcn=sps_rtmsupport('CopyFcn',gcbh); powericon('ThreePhaseVIMeasurementCopy',gcb)  DeleteFcn=sps_rtmsupport('DeleteFcn',gcbh);  UndoDeleteFcn=sps_rtmsupport('UndoDeleteFcn',gcbh);  ModelCloseFcn=sps_rtmsupport('ModelCloseFcn',gcbh);  PreSaveFcn="sps_rtmsupport('PreSaveFcn',gcbh);  set_param(gcb,'LinkStatus','restore')"  PostSaveFcn=sps_rtmsupport('PostSaveFcn',gcbh);  NameChangeFcn=sps_rtmsupport('NameChangeFcn',gcbh);  PreCopyFcn=sps_rtmsupport('PreCopyFcn',gcbh);  OpenFcn=sps_rtmsupport('OpenFcn',gcbh, [1 2 4 5 6 7 9 -12 13]);  CloseFcn=sps_rtmsupport('CloseFcn',gcbh);  PreDeleteFcn=sps_rtmsupport('PreDeleteFcn',gcbh);
      mask Help: helpview(psbhelp)
      mask TypeOptions VoltageMeasurement: no | phase-to-ground | phase-to-phase
      mask Callback VoltageMeasurement: powericon('ThreePhaseVIMeasurementCback',gcb,'Vselector');
      mask Callback SetLabelV: powericon('ThreePhaseVIMeasurementCback',gcb,'');
      mask Callback Vpu: powericon('ThreePhaseVIMeasurementCback',gcb,'Vpu');
      mask Callback VpuLL: powericon('ThreePhaseVIMeasurementCback',gcb,'VpuLL');
      mask TypeOptions CurrentMeasurement: no | yes
      mask Callback CurrentMeasurement: powericon('ThreePhaseVIMeasurementCback',gcb,'');
      mask Callback SetLabelI: powericon('ThreePhaseVIMeasurementCback',gcb,'');
      mask Callback LabelI: powericon('ThreePhaseVIMeasurementCback',gcb,'');
      mask Callback Ipu: powericon('ThreePhaseVIMeasurementCback',gcb,'');
      mask TypeOptions OutputType: Complex | Real-Imag | Magnitude-Angle | Magnitude
  BusC17 : Subsystem  DialogController=POWERSYS.PowerSysDialog  LoadFcn=sps_rtmsupport('LoadFcn',gcbh);  StartFcn=sps_rtmsupport('StartFcn',gcbh);  StopFcn=sps_rtmsupport('StopFcn',gcbh);  mask(Three-Phase VI Measurement){VoltageMeasurement=phase-to-ground, SetLabelV=off, LabelV=Vabc, Vpu=off, VpuLL=off, CurrentMeasurement=yes, SetLabelI=off, LabelI=Iabc, Ipu=off, Pbase=100e6, Vbase=500e3, OutputType=Complex, PhasorSimulation=off, PSBequivalent=0}
      mask prompts: VoltageMeasurement "Voltage measurement"; SetLabelV "Use a label"; LabelV "Signal label  (use a From block to collect this signal)"; Vpu "Voltages in pu,  based on peak value of nominal phase-to-ground voltage"; VpuLL "Voltages in pu,  based on peak value of nominal phase-to-phase  voltage"; CurrentMeasurement "Current measurement"; SetLabelI "Use a label"; LabelI "Signal label  (use a From block to collect this signal)"; Ipu "Currents in pu"; Pbase "Base power ( VA 3 phase)"; Vbase "Nominal voltage used for pu measurement (Vrms phase-phase) :"; OutputType "Output signals in:"; PhasorSimulation "Phasor simulation (internal use)"; PSBequivalent "Equivalent circuit (internal use)"
      mask help:
      | Ideal three-phase voltage and current measurements.
      |
      | The block can output the voltages and currents in per unit values or in volts and amperes.
      mask init: same as Versie2/SM_WT1/BusA
      settings: CopyFcn=sps_rtmsupport('CopyFcn',gcbh); powericon('ThreePhaseVIMeasurementCopy',gcb)  DeleteFcn=sps_rtmsupport('DeleteFcn',gcbh);  UndoDeleteFcn=sps_rtmsupport('UndoDeleteFcn',gcbh);  ModelCloseFcn=sps_rtmsupport('ModelCloseFcn',gcbh);  PreSaveFcn="sps_rtmsupport('PreSaveFcn',gcbh);  set_param(gcb,'LinkStatus','restore')"  PostSaveFcn=sps_rtmsupport('PostSaveFcn',gcbh);  NameChangeFcn=sps_rtmsupport('NameChangeFcn',gcbh);  PreCopyFcn=sps_rtmsupport('PreCopyFcn',gcbh);  OpenFcn=sps_rtmsupport('OpenFcn',gcbh, [1 2 4 5 6 7 9 -12 13]);  CloseFcn=sps_rtmsupport('CloseFcn',gcbh);  PreDeleteFcn=sps_rtmsupport('PreDeleteFcn',gcbh);
      mask Help: helpview(psbhelp)
      mask TypeOptions VoltageMeasurement: no | phase-to-ground | phase-to-phase
      mask Callback VoltageMeasurement: powericon('ThreePhaseVIMeasurementCback',gcb,'Vselector');
      mask Callback SetLabelV: powericon('ThreePhaseVIMeasurementCback',gcb,'');
      mask Callback Vpu: powericon('ThreePhaseVIMeasurementCback',gcb,'Vpu');
      mask Callback VpuLL: powericon('ThreePhaseVIMeasurementCback',gcb,'VpuLL');
      mask TypeOptions CurrentMeasurement: no | yes
      mask Callback CurrentMeasurement: powericon('ThreePhaseVIMeasurementCback',gcb,'');
      mask Callback SetLabelI: powericon('ThreePhaseVIMeasurementCback',gcb,'');
      mask Callback LabelI: powericon('ThreePhaseVIMeasurementCback',gcb,'');
      mask Callback Ipu: powericon('ThreePhaseVIMeasurementCback',gcb,'');
      mask TypeOptions OutputType: Complex | Real-Imag | Magnitude-Angle | Magnitude
  BusC2 : Subsystem  DialogController=POWERSYS.PowerSysDialog  LoadFcn=sps_rtmsupport('LoadFcn',gcbh);  StartFcn=sps_rtmsupport('StartFcn',gcbh);  StopFcn=sps_rtmsupport('StopFcn',gcbh);  mask(Three-Phase VI Measurement){VoltageMeasurement=phase-to-ground, SetLabelV=off, LabelV=Vabc, Vpu=off, VpuLL=off, CurrentMeasurement=yes, SetLabelI=off, LabelI=Iabc, Ipu=off, Pbase=100e6, Vbase=500e3, OutputType=Complex, PhasorSimulation=off, PSBequivalent=0}
      mask prompts: VoltageMeasurement "Voltage measurement"; SetLabelV "Use a label"; LabelV "Signal label  (use a From block to collect this signal)"; Vpu "Voltages in pu,  based on peak value of nominal phase-to-ground voltage"; VpuLL "Voltages in pu,  based on peak value of nominal phase-to-phase  voltage"; CurrentMeasurement "Current measurement"; SetLabelI "Use a label"; LabelI "Signal label  (use a From block to collect this signal)"; Ipu "Currents in pu"; Pbase "Base power ( VA 3 phase)"; Vbase "Nominal voltage used for pu measurement (Vrms phase-phase) :"; OutputType "Output signals in:"; PhasorSimulation "Phasor simulation (internal use)"; PSBequivalent "Equivalent circuit (internal use)"
      mask help:
      | Ideal three-phase voltage and current measurements.
      |
      | The block can output the voltages and currents in per unit values or in volts and amperes.
      mask init: same as Versie2/SM_WT1/BusA
      settings: CopyFcn=sps_rtmsupport('CopyFcn',gcbh); powericon('ThreePhaseVIMeasurementCopy',gcb)  DeleteFcn=sps_rtmsupport('DeleteFcn',gcbh);  UndoDeleteFcn=sps_rtmsupport('UndoDeleteFcn',gcbh);  ModelCloseFcn=sps_rtmsupport('ModelCloseFcn',gcbh);  PreSaveFcn="sps_rtmsupport('PreSaveFcn',gcbh);  set_param(gcb,'LinkStatus','restore')"  PostSaveFcn=sps_rtmsupport('PostSaveFcn',gcbh);  NameChangeFcn=sps_rtmsupport('NameChangeFcn',gcbh);  PreCopyFcn=sps_rtmsupport('PreCopyFcn',gcbh);  OpenFcn=sps_rtmsupport('OpenFcn',gcbh, [1 2 4 5 6 7 9 -12 13]);  CloseFcn=sps_rtmsupport('CloseFcn',gcbh);  PreDeleteFcn=sps_rtmsupport('PreDeleteFcn',gcbh);
      mask Help: helpview(psbhelp)
      mask TypeOptions VoltageMeasurement: no | phase-to-ground | phase-to-phase
      mask Callback VoltageMeasurement: powericon('ThreePhaseVIMeasurementCback',gcb,'Vselector');
      mask Callback SetLabelV: powericon('ThreePhaseVIMeasurementCback',gcb,'');
      mask Callback Vpu: powericon('ThreePhaseVIMeasurementCback',gcb,'Vpu');
      mask Callback VpuLL: powericon('ThreePhaseVIMeasurementCback',gcb,'VpuLL');
      mask TypeOptions CurrentMeasurement: no | yes
      mask Callback CurrentMeasurement: powericon('ThreePhaseVIMeasurementCback',gcb,'');
      mask Callback SetLabelI: powericon('ThreePhaseVIMeasurementCback',gcb,'');
      mask Callback LabelI: powericon('ThreePhaseVIMeasurementCback',gcb,'');
      mask Callback Ipu: powericon('ThreePhaseVIMeasurementCback',gcb,'');
      mask TypeOptions OutputType: Complex | Real-Imag | Magnitude-Angle | Magnitude
  BusC3 : Subsystem  DialogController=POWERSYS.PowerSysDialog  LoadFcn=sps_rtmsupport('LoadFcn',gcbh);  StartFcn=sps_rtmsupport('StartFcn',gcbh);  StopFcn=sps_rtmsupport('StopFcn',gcbh);  mask(Three-Phase VI Measurement){VoltageMeasurement=phase-to-ground, SetLabelV=off, LabelV=Vabc, Vpu=off, VpuLL=off, CurrentMeasurement=yes, SetLabelI=off, LabelI=Iabc, Ipu=off, Pbase=100e6, Vbase=500e3, OutputType=Complex, PhasorSimulation=off, PSBequivalent=0}
      mask prompts: VoltageMeasurement "Voltage measurement"; SetLabelV "Use a label"; LabelV "Signal label  (use a From block to collect this signal)"; Vpu "Voltages in pu,  based on peak value of nominal phase-to-ground voltage"; VpuLL "Voltages in pu,  based on peak value of nominal phase-to-phase  voltage"; CurrentMeasurement "Current measurement"; SetLabelI "Use a label"; LabelI "Signal label  (use a From block to collect this signal)"; Ipu "Currents in pu"; Pbase "Base power ( VA 3 phase)"; Vbase "Nominal voltage used for pu measurement (Vrms phase-phase) :"; OutputType "Output signals in:"; PhasorSimulation "Phasor simulation (internal use)"; PSBequivalent "Equivalent circuit (internal use)"
      mask help:
      | Ideal three-phase voltage and current measurements.
      |
      | The block can output the voltages and currents in per unit values or in volts and amperes.
      mask init: same as Versie2/SM_WT1/BusA
      settings: CopyFcn=sps_rtmsupport('CopyFcn',gcbh); powericon('ThreePhaseVIMeasurementCopy',gcb)  DeleteFcn=sps_rtmsupport('DeleteFcn',gcbh);  UndoDeleteFcn=sps_rtmsupport('UndoDeleteFcn',gcbh);  ModelCloseFcn=sps_rtmsupport('ModelCloseFcn',gcbh);  PreSaveFcn="sps_rtmsupport('PreSaveFcn',gcbh);  set_param(gcb,'LinkStatus','restore')"  PostSaveFcn=sps_rtmsupport('PostSaveFcn',gcbh);  NameChangeFcn=sps_rtmsupport('NameChangeFcn',gcbh);  PreCopyFcn=sps_rtmsupport('PreCopyFcn',gcbh);  OpenFcn=sps_rtmsupport('OpenFcn',gcbh, [1 2 4 5 6 7 9 -12 13]);  CloseFcn=sps_rtmsupport('CloseFcn',gcbh);  PreDeleteFcn=sps_rtmsupport('PreDeleteFcn',gcbh);
      mask Help: helpview(psbhelp)
      mask TypeOptions VoltageMeasurement: no | phase-to-ground | phase-to-phase
      mask Callback VoltageMeasurement: powericon('ThreePhaseVIMeasurementCback',gcb,'Vselector');
      mask Callback SetLabelV: powericon('ThreePhaseVIMeasurementCback',gcb,'');
      mask Callback Vpu: powericon('ThreePhaseVIMeasurementCback',gcb,'Vpu');
      mask Callback VpuLL: powericon('ThreePhaseVIMeasurementCback',gcb,'VpuLL');
      mask TypeOptions CurrentMeasurement: no | yes
      mask Callback CurrentMeasurement: powericon('ThreePhaseVIMeasurementCback',gcb,'');
      mask Callback SetLabelI: powericon('ThreePhaseVIMeasurementCback',gcb,'');
      mask Callback LabelI: powericon('ThreePhaseVIMeasurementCback',gcb,'');
      mask Callback Ipu: powericon('ThreePhaseVIMeasurementCback',gcb,'');
      mask TypeOptions OutputType: Complex | Real-Imag | Magnitude-Angle | Magnitude
  BusC4 : Subsystem  DialogController=POWERSYS.PowerSysDialog  LoadFcn=sps_rtmsupport('LoadFcn',gcbh);  StartFcn=sps_rtmsupport('StartFcn',gcbh);  StopFcn=sps_rtmsupport('StopFcn',gcbh);  mask(Three-Phase VI Measurement){VoltageMeasurement=phase-to-ground, SetLabelV=off, LabelV=Vabc, Vpu=off, VpuLL=off, CurrentMeasurement=yes, SetLabelI=off, LabelI=Iabc, Ipu=off, Pbase=100e6, Vbase=500e3, OutputType=Complex, PhasorSimulation=off, PSBequivalent=0}
      mask prompts: VoltageMeasurement "Voltage measurement"; SetLabelV "Use a label"; LabelV "Signal label  (use a From block to collect this signal)"; Vpu "Voltages in pu,  based on peak value of nominal phase-to-ground voltage"; VpuLL "Voltages in pu,  based on peak value of nominal phase-to-phase  voltage"; CurrentMeasurement "Current measurement"; SetLabelI "Use a label"; LabelI "Signal label  (use a From block to collect this signal)"; Ipu "Currents in pu"; Pbase "Base power ( VA 3 phase)"; Vbase "Nominal voltage used for pu measurement (Vrms phase-phase) :"; OutputType "Output signals in:"; PhasorSimulation "Phasor simulation (internal use)"; PSBequivalent "Equivalent circuit (internal use)"
      mask help:
      | Ideal three-phase voltage and current measurements.
      |
      | The block can output the voltages and currents in per unit values or in volts and amperes.
      mask init: same as Versie2/SM_WT1/BusA
      settings: CopyFcn=sps_rtmsupport('CopyFcn',gcbh); powericon('ThreePhaseVIMeasurementCopy',gcb)  DeleteFcn=sps_rtmsupport('DeleteFcn',gcbh);  UndoDeleteFcn=sps_rtmsupport('UndoDeleteFcn',gcbh);  ModelCloseFcn=sps_rtmsupport('ModelCloseFcn',gcbh);  PreSaveFcn="sps_rtmsupport('PreSaveFcn',gcbh);  set_param(gcb,'LinkStatus','restore')"  PostSaveFcn=sps_rtmsupport('PostSaveFcn',gcbh);  NameChangeFcn=sps_rtmsupport('NameChangeFcn',gcbh);  PreCopyFcn=sps_rtmsupport('PreCopyFcn',gcbh);  OpenFcn=sps_rtmsupport('OpenFcn',gcbh, [1 2 4 5 6 7 9 -12 13]);  CloseFcn=sps_rtmsupport('CloseFcn',gcbh);  PreDeleteFcn=sps_rtmsupport('PreDeleteFcn',gcbh);
      mask Help: helpview(psbhelp)
      mask TypeOptions VoltageMeasurement: no | phase-to-ground | phase-to-phase
      mask Callback VoltageMeasurement: powericon('ThreePhaseVIMeasurementCback',gcb,'Vselector');
      mask Callback SetLabelV: powericon('ThreePhaseVIMeasurementCback',gcb,'');
      mask Callback Vpu: powericon('ThreePhaseVIMeasurementCback',gcb,'Vpu');
      mask Callback VpuLL: powericon('ThreePhaseVIMeasurementCback',gcb,'VpuLL');
      mask TypeOptions CurrentMeasurement: no | yes
      mask Callback CurrentMeasurement: powericon('ThreePhaseVIMeasurementCback',gcb,'');
      mask Callback SetLabelI: powericon('ThreePhaseVIMeasurementCback',gcb,'');
      mask Callback LabelI: powericon('ThreePhaseVIMeasurementCback',gcb,'');
      mask Callback Ipu: powericon('ThreePhaseVIMeasurementCback',gcb,'');
      mask TypeOptions OutputType: Complex | Real-Imag | Magnitude-Angle | Magnitude
  BusC5 : Subsystem  DialogController=POWERSYS.PowerSysDialog  LoadFcn=sps_rtmsupport('LoadFcn',gcbh);  StartFcn=sps_rtmsupport('StartFcn',gcbh);  StopFcn=sps_rtmsupport('StopFcn',gcbh);  mask(Three-Phase VI Measurement){VoltageMeasurement=phase-to-ground, SetLabelV=off, LabelV=Vabc, Vpu=off, VpuLL=off, CurrentMeasurement=yes, SetLabelI=off, LabelI=Iabc, Ipu=off, Pbase=100e6, Vbase=500e3, OutputType=Complex, PhasorSimulation=off, PSBequivalent=0}
      mask prompts: VoltageMeasurement "Voltage measurement"; SetLabelV "Use a label"; LabelV "Signal label  (use a From block to collect this signal)"; Vpu "Voltages in pu,  based on peak value of nominal phase-to-ground voltage"; VpuLL "Voltages in pu,  based on peak value of nominal phase-to-phase  voltage"; CurrentMeasurement "Current measurement"; SetLabelI "Use a label"; LabelI "Signal label  (use a From block to collect this signal)"; Ipu "Currents in pu"; Pbase "Base power ( VA 3 phase)"; Vbase "Nominal voltage used for pu measurement (Vrms phase-phase) :"; OutputType "Output signals in:"; PhasorSimulation "Phasor simulation (internal use)"; PSBequivalent "Equivalent circuit (internal use)"
      mask help:
      | Ideal three-phase voltage and current measurements.
      |
      | The block can output the voltages and currents in per unit values or in volts and amperes.
      mask init: same as Versie2/SM_WT1/BusA
      settings: CopyFcn=sps_rtmsupport('CopyFcn',gcbh); powericon('ThreePhaseVIMeasurementCopy',gcb)  DeleteFcn=sps_rtmsupport('DeleteFcn',gcbh);  UndoDeleteFcn=sps_rtmsupport('UndoDeleteFcn',gcbh);  ModelCloseFcn=sps_rtmsupport('ModelCloseFcn',gcbh);  PreSaveFcn="sps_rtmsupport('PreSaveFcn',gcbh);  set_param(gcb,'LinkStatus','restore')"  PostSaveFcn=sps_rtmsupport('PostSaveFcn',gcbh);  NameChangeFcn=sps_rtmsupport('NameChangeFcn',gcbh);  PreCopyFcn=sps_rtmsupport('PreCopyFcn',gcbh);  OpenFcn=sps_rtmsupport('OpenFcn',gcbh, [1 2 4 5 6 7 9 -12 13]);  CloseFcn=sps_rtmsupport('CloseFcn',gcbh);  PreDeleteFcn=sps_rtmsupport('PreDeleteFcn',gcbh);
      mask Help: helpview(psbhelp)
      mask TypeOptions VoltageMeasurement: no | phase-to-ground | phase-to-phase
      mask Callback VoltageMeasurement: powericon('ThreePhaseVIMeasurementCback',gcb,'Vselector');
      mask Callback SetLabelV: powericon('ThreePhaseVIMeasurementCback',gcb,'');
      mask Callback Vpu: powericon('ThreePhaseVIMeasurementCback',gcb,'Vpu');
      mask Callback VpuLL: powericon('ThreePhaseVIMeasurementCback',gcb,'VpuLL');
      mask TypeOptions CurrentMeasurement: no | yes
      mask Callback CurrentMeasurement: powericon('ThreePhaseVIMeasurementCback',gcb,'');
      mask Callback SetLabelI: powericon('ThreePhaseVIMeasurementCback',gcb,'');
      mask Callback LabelI: powericon('ThreePhaseVIMeasurementCback',gcb,'');
      mask Callback Ipu: powericon('ThreePhaseVIMeasurementCback',gcb,'');
      mask TypeOptions OutputType: Complex | Real-Imag | Magnitude-Angle | Magnitude
  BusC6 : Subsystem  DialogController=POWERSYS.PowerSysDialog  LoadFcn=sps_rtmsupport('LoadFcn',gcbh);  StartFcn=sps_rtmsupport('StartFcn',gcbh);  StopFcn=sps_rtmsupport('StopFcn',gcbh);  mask(Three-Phase VI Measurement){VoltageMeasurement=phase-to-ground, SetLabelV=off, LabelV=Vabc, Vpu=off, VpuLL=off, CurrentMeasurement=yes, SetLabelI=off, LabelI=Iabc, Ipu=off, Pbase=100e6, Vbase=500e3, OutputType=Complex, PhasorSimulation=off, PSBequivalent=0}
      mask prompts: VoltageMeasurement "Voltage measurement"; SetLabelV "Use a label"; LabelV "Signal label  (use a From block to collect this signal)"; Vpu "Voltages in pu,  based on peak value of nominal phase-to-ground voltage"; VpuLL "Voltages in pu,  based on peak value of nominal phase-to-phase  voltage"; CurrentMeasurement "Current measurement"; SetLabelI "Use a label"; LabelI "Signal label  (use a From block to collect this signal)"; Ipu "Currents in pu"; Pbase "Base power ( VA 3 phase)"; Vbase "Nominal voltage used for pu measurement (Vrms phase-phase) :"; OutputType "Output signals in:"; PhasorSimulation "Phasor simulation (internal use)"; PSBequivalent "Equivalent circuit (internal use)"
      mask help:
      | Ideal three-phase voltage and current measurements.
      |
      | The block can output the voltages and currents in per unit values or in volts and amperes.
      mask init: same as Versie2/SM_WT1/BusA
      settings: CopyFcn=sps_rtmsupport('CopyFcn',gcbh); powericon('ThreePhaseVIMeasurementCopy',gcb)  DeleteFcn=sps_rtmsupport('DeleteFcn',gcbh);  UndoDeleteFcn=sps_rtmsupport('UndoDeleteFcn',gcbh);  ModelCloseFcn=sps_rtmsupport('ModelCloseFcn',gcbh);  PreSaveFcn="sps_rtmsupport('PreSaveFcn',gcbh);  set_param(gcb,'LinkStatus','restore')"  PostSaveFcn=sps_rtmsupport('PostSaveFcn',gcbh);  NameChangeFcn=sps_rtmsupport('NameChangeFcn',gcbh);  PreCopyFcn=sps_rtmsupport('PreCopyFcn',gcbh);  OpenFcn=sps_rtmsupport('OpenFcn',gcbh, [1 2 4 5 6 7 9 -12 13]);  CloseFcn=sps_rtmsupport('CloseFcn',gcbh);  PreDeleteFcn=sps_rtmsupport('PreDeleteFcn',gcbh);
      mask Help: helpview(psbhelp)
      mask TypeOptions VoltageMeasurement: no | phase-to-ground | phase-to-phase
      mask Callback VoltageMeasurement: powericon('ThreePhaseVIMeasurementCback',gcb,'Vselector');
      mask Callback SetLabelV: powericon('ThreePhaseVIMeasurementCback',gcb,'');
      mask Callback Vpu: powericon('ThreePhaseVIMeasurementCback',gcb,'Vpu');
      mask Callback VpuLL: powericon('ThreePhaseVIMeasurementCback',gcb,'VpuLL');
      mask TypeOptions CurrentMeasurement: no | yes
      mask Callback CurrentMeasurement: powericon('ThreePhaseVIMeasurementCback',gcb,'');
      mask Callback SetLabelI: powericon('ThreePhaseVIMeasurementCback',gcb,'');
      mask Callback LabelI: powericon('ThreePhaseVIMeasurementCback',gcb,'');
      mask Callback Ipu: powericon('ThreePhaseVIMeasurementCback',gcb,'');
      mask TypeOptions OutputType: Complex | Real-Imag | Magnitude-Angle | Magnitude
  BusC7 : Subsystem  DialogController=POWERSYS.PowerSysDialog  LoadFcn=sps_rtmsupport('LoadFcn',gcbh);  StartFcn=sps_rtmsupport('StartFcn',gcbh);  StopFcn=sps_rtmsupport('StopFcn',gcbh);  mask(Three-Phase VI Measurement){VoltageMeasurement=phase-to-ground, SetLabelV=off, LabelV=Vabc, Vpu=off, VpuLL=off, CurrentMeasurement=yes, SetLabelI=off, LabelI=Iabc, Ipu=off, Pbase=100e6, Vbase=500e3, OutputType=Complex, PhasorSimulation=off, PSBequivalent=0}
      mask prompts: VoltageMeasurement "Voltage measurement"; SetLabelV "Use a label"; LabelV "Signal label  (use a From block to collect this signal)"; Vpu "Voltages in pu,  based on peak value of nominal phase-to-ground voltage"; VpuLL "Voltages in pu,  based on peak value of nominal phase-to-phase  voltage"; CurrentMeasurement "Current measurement"; SetLabelI "Use a label"; LabelI "Signal label  (use a From block to collect this signal)"; Ipu "Currents in pu"; Pbase "Base power ( VA 3 phase)"; Vbase "Nominal voltage used for pu measurement (Vrms phase-phase) :"; OutputType "Output signals in:"; PhasorSimulation "Phasor simulation (internal use)"; PSBequivalent "Equivalent circuit (internal use)"
      mask help:
      | Ideal three-phase voltage and current measurements.
      |
      | The block can output the voltages and currents in per unit values or in volts and amperes.
      mask init: same as Versie2/SM_WT1/BusA
      settings: CopyFcn=sps_rtmsupport('CopyFcn',gcbh); powericon('ThreePhaseVIMeasurementCopy',gcb)  DeleteFcn=sps_rtmsupport('DeleteFcn',gcbh);  UndoDeleteFcn=sps_rtmsupport('UndoDeleteFcn',gcbh);  ModelCloseFcn=sps_rtmsupport('ModelCloseFcn',gcbh);  PreSaveFcn="sps_rtmsupport('PreSaveFcn',gcbh);  set_param(gcb,'LinkStatus','restore')"  PostSaveFcn=sps_rtmsupport('PostSaveFcn',gcbh);  NameChangeFcn=sps_rtmsupport('NameChangeFcn',gcbh);  PreCopyFcn=sps_rtmsupport('PreCopyFcn',gcbh);  OpenFcn=sps_rtmsupport('OpenFcn',gcbh, [1 2 4 5 6 7 9 -12 13]);  CloseFcn=sps_rtmsupport('CloseFcn',gcbh);  PreDeleteFcn=sps_rtmsupport('PreDeleteFcn',gcbh);
      mask Help: helpview(psbhelp)
      mask TypeOptions VoltageMeasurement: no | phase-to-ground | phase-to-phase
      mask Callback VoltageMeasurement: powericon('ThreePhaseVIMeasurementCback',gcb,'Vselector');
      mask Callback SetLabelV: powericon('ThreePhaseVIMeasurementCback',gcb,'');
      mask Callback Vpu: powericon('ThreePhaseVIMeasurementCback',gcb,'Vpu');
      mask Callback VpuLL: powericon('ThreePhaseVIMeasurementCback',gcb,'VpuLL');
      mask TypeOptions CurrentMeasurement: no | yes
      mask Callback CurrentMeasurement: powericon('ThreePhaseVIMeasurementCback',gcb,'');
      mask Callback SetLabelI: powericon('ThreePhaseVIMeasurementCback',gcb,'');
      mask Callback LabelI: powericon('ThreePhaseVIMeasurementCback',gcb,'');
      mask Callback Ipu: powericon('ThreePhaseVIMeasurementCback',gcb,'');
      mask TypeOptions OutputType: Complex | Real-Imag | Magnitude-Angle | Magnitude
  BusC8 : Subsystem  DialogController=POWERSYS.PowerSysDialog  LoadFcn=sps_rtmsupport('LoadFcn',gcbh);  StartFcn=sps_rtmsupport('StartFcn',gcbh);  StopFcn=sps_rtmsupport('StopFcn',gcbh);  mask(Three-Phase VI Measurement){VoltageMeasurement=phase-to-ground, SetLabelV=off, LabelV=Vabc, Vpu=off, VpuLL=off, CurrentMeasurement=yes, SetLabelI=off, LabelI=Iabc, Ipu=off, Pbase=100e6, Vbase=500e3, OutputType=Complex, PhasorSimulation=off, PSBequivalent=0}
      mask prompts: VoltageMeasurement "Voltage measurement"; SetLabelV "Use a label"; LabelV "Signal label  (use a From block to collect this signal)"; Vpu "Voltages in pu,  based on peak value of nominal phase-to-ground voltage"; VpuLL "Voltages in pu,  based on peak value of nominal phase-to-phase  voltage"; CurrentMeasurement "Current measurement"; SetLabelI "Use a label"; LabelI "Signal label  (use a From block to collect this signal)"; Ipu "Currents in pu"; Pbase "Base power ( VA 3 phase)"; Vbase "Nominal voltage used for pu measurement (Vrms phase-phase) :"; OutputType "Output signals in:"; PhasorSimulation "Phasor simulation (internal use)"; PSBequivalent "Equivalent circuit (internal use)"
      mask help:
      | Ideal three-phase voltage and current measurements.
      |
      | The block can output the voltages and currents in per unit values or in volts and amperes.
      mask init: same as Versie2/SM_WT1/BusA
      settings: CopyFcn=sps_rtmsupport('CopyFcn',gcbh); powericon('ThreePhaseVIMeasurementCopy',gcb)  DeleteFcn=sps_rtmsupport('DeleteFcn',gcbh);  UndoDeleteFcn=sps_rtmsupport('UndoDeleteFcn',gcbh);  ModelCloseFcn=sps_rtmsupport('ModelCloseFcn',gcbh);  PreSaveFcn="sps_rtmsupport('PreSaveFcn',gcbh);  set_param(gcb,'LinkStatus','restore')"  PostSaveFcn=sps_rtmsupport('PostSaveFcn',gcbh);  NameChangeFcn=sps_rtmsupport('NameChangeFcn',gcbh);  PreCopyFcn=sps_rtmsupport('PreCopyFcn',gcbh);  OpenFcn=sps_rtmsupport('OpenFcn',gcbh, [1 2 4 5 6 7 9 -12 13]);  CloseFcn=sps_rtmsupport('CloseFcn',gcbh);  PreDeleteFcn=sps_rtmsupport('PreDeleteFcn',gcbh);
      mask Help: helpview(psbhelp)
      mask TypeOptions VoltageMeasurement: no | phase-to-ground | phase-to-phase
      mask Callback VoltageMeasurement: powericon('ThreePhaseVIMeasurementCback',gcb,'Vselector');
      mask Callback SetLabelV: powericon('ThreePhaseVIMeasurementCback',gcb,'');
      mask Callback Vpu: powericon('ThreePhaseVIMeasurementCback',gcb,'Vpu');
      mask Callback VpuLL: powericon('ThreePhaseVIMeasurementCback',gcb,'VpuLL');
      mask TypeOptions CurrentMeasurement: no | yes
      mask Callback CurrentMeasurement: powericon('ThreePhaseVIMeasurementCback',gcb,'');
      mask Callback SetLabelI: powericon('ThreePhaseVIMeasurementCback',gcb,'');
      mask Callback LabelI: powericon('ThreePhaseVIMeasurementCback',gcb,'');
      mask Callback Ipu: powericon('ThreePhaseVIMeasurementCback',gcb,'');
      mask TypeOptions OutputType: Complex | Real-Imag | Magnitude-Angle | Magnitude
  BusC9 : Subsystem  DialogController=POWERSYS.PowerSysDialog  LoadFcn=sps_rtmsupport('LoadFcn',gcbh);  StartFcn=sps_rtmsupport('StartFcn',gcbh);  StopFcn=sps_rtmsupport('StopFcn',gcbh);  mask(Three-Phase VI Measurement){VoltageMeasurement=phase-to-ground, SetLabelV=off, LabelV=Vabc, Vpu=off, VpuLL=off, CurrentMeasurement=yes, SetLabelI=off, LabelI=Iabc, Ipu=off, Pbase=100e6, Vbase=500e3, OutputType=Complex, PhasorSimulation=off, PSBequivalent=0}
      mask prompts: VoltageMeasurement "Voltage measurement"; SetLabelV "Use a label"; LabelV "Signal label  (use a From block to collect this signal)"; Vpu "Voltages in pu,  based on peak value of nominal phase-to-ground voltage"; VpuLL "Voltages in pu,  based on peak value of nominal phase-to-phase  voltage"; CurrentMeasurement "Current measurement"; SetLabelI "Use a label"; LabelI "Signal label  (use a From block to collect this signal)"; Ipu "Currents in pu"; Pbase "Base power ( VA 3 phase)"; Vbase "Nominal voltage used for pu measurement (Vrms phase-phase) :"; OutputType "Output signals in:"; PhasorSimulation "Phasor simulation (internal use)"; PSBequivalent "Equivalent circuit (internal use)"
      mask help:
      | Ideal three-phase voltage and current measurements.
      |
      | The block can output the voltages and currents in per unit values or in volts and amperes.
      mask init: same as Versie2/SM_WT1/BusA
      settings: CopyFcn=sps_rtmsupport('CopyFcn',gcbh); powericon('ThreePhaseVIMeasurementCopy',gcb)  DeleteFcn=sps_rtmsupport('DeleteFcn',gcbh);  UndoDeleteFcn=sps_rtmsupport('UndoDeleteFcn',gcbh);  ModelCloseFcn=sps_rtmsupport('ModelCloseFcn',gcbh);  PreSaveFcn="sps_rtmsupport('PreSaveFcn',gcbh);  set_param(gcb,'LinkStatus','restore')"  PostSaveFcn=sps_rtmsupport('PostSaveFcn',gcbh);  NameChangeFcn=sps_rtmsupport('NameChangeFcn',gcbh);  PreCopyFcn=sps_rtmsupport('PreCopyFcn',gcbh);  OpenFcn=sps_rtmsupport('OpenFcn',gcbh, [1 2 4 5 6 7 9 -12 13]);  CloseFcn=sps_rtmsupport('CloseFcn',gcbh);  PreDeleteFcn=sps_rtmsupport('PreDeleteFcn',gcbh);
      mask Help: helpview(psbhelp)
      mask TypeOptions VoltageMeasurement: no | phase-to-ground | phase-to-phase
      mask Callback VoltageMeasurement: powericon('ThreePhaseVIMeasurementCback',gcb,'Vselector');
      mask Callback SetLabelV: powericon('ThreePhaseVIMeasurementCback',gcb,'');
      mask Callback Vpu: powericon('ThreePhaseVIMeasurementCback',gcb,'Vpu');
      mask Callback VpuLL: powericon('ThreePhaseVIMeasurementCback',gcb,'VpuLL');
      mask TypeOptions CurrentMeasurement: no | yes
      mask Callback CurrentMeasurement: powericon('ThreePhaseVIMeasurementCback',gcb,'');
      mask Callback SetLabelI: powericon('ThreePhaseVIMeasurementCback',gcb,'');
      mask Callback LabelI: powericon('ThreePhaseVIMeasurementCback',gcb,'');
      mask Callback Ipu: powericon('ThreePhaseVIMeasurementCback',gcb,'');
      mask TypeOptions OutputType: Complex | Real-Imag | Magnitude-Angle | Magnitude
  BusD : Subsystem  Commented=on  DialogController=POWERSYS.PowerSysDialog  LoadFcn=sps_rtmsupport('LoadFcn',gcbh);  StartFcn=sps_rtmsupport('StartFcn',gcbh);  StopFcn=sps_rtmsupport('StopFcn',gcbh);  mask(Three-Phase VI Measurement){VoltageMeasurement=phase-to-ground, SetLabelV=off, LabelV=Vabc, Vpu=off, VpuLL=off, CurrentMeasurement=yes, SetLabelI=off, LabelI=Iabc, Ipu=off, Pbase=100e6, Vbase=500e3, OutputType=Complex, PhasorSimulation=off, PSBequivalent=0}
      mask prompts: VoltageMeasurement "Voltage measurement"; SetLabelV "Use a label"; LabelV "Signal label  (use a From block to collect this signal)"; Vpu "Voltages in pu,  based on peak value of nominal phase-to-ground voltage"; VpuLL "Voltages in pu,  based on peak value of nominal phase-to-phase  voltage"; CurrentMeasurement "Current measurement"; SetLabelI "Use a label"; LabelI "Signal label  (use a From block to collect this signal)"; Ipu "Currents in pu"; Pbase "Base power ( VA 3 phase)"; Vbase "Nominal voltage used for pu measurement (Vrms phase-phase) :"; OutputType "Output signals in:"; PhasorSimulation "Phasor simulation (internal use)"; PSBequivalent "Equivalent circuit (internal use)"
      mask help:
      | Ideal three-phase voltage and current measurements.
      |
      | The block can output the voltages and currents in per unit values or in volts and amperes.
      mask init: same as Versie2/SM_WT1/BusA
      settings: CopyFcn=sps_rtmsupport('CopyFcn',gcbh); powericon('ThreePhaseVIMeasurementCopy',gcb)  DeleteFcn=sps_rtmsupport('DeleteFcn',gcbh);  UndoDeleteFcn=sps_rtmsupport('UndoDeleteFcn',gcbh);  ModelCloseFcn=sps_rtmsupport('ModelCloseFcn',gcbh);  PreSaveFcn="sps_rtmsupport('PreSaveFcn',gcbh);  set_param(gcb,'LinkStatus','restore')"  PostSaveFcn=sps_rtmsupport('PostSaveFcn',gcbh);  NameChangeFcn=sps_rtmsupport('NameChangeFcn',gcbh);  PreCopyFcn=sps_rtmsupport('PreCopyFcn',gcbh);  OpenFcn=sps_rtmsupport('OpenFcn',gcbh, [1 2 4 5 6 7 9 -12 13]);  CloseFcn=sps_rtmsupport('CloseFcn',gcbh);  PreDeleteFcn=sps_rtmsupport('PreDeleteFcn',gcbh);
      mask Help: helpview(psbhelp)
      mask TypeOptions VoltageMeasurement: no | phase-to-ground | phase-to-phase
      mask Callback VoltageMeasurement: powericon('ThreePhaseVIMeasurementCback',gcb,'Vselector');
      mask Callback SetLabelV: powericon('ThreePhaseVIMeasurementCback',gcb,'');
      mask Callback Vpu: powericon('ThreePhaseVIMeasurementCback',gcb,'Vpu');
      mask Callback VpuLL: powericon('ThreePhaseVIMeasurementCback',gcb,'VpuLL');
      mask TypeOptions CurrentMeasurement: no | yes
      mask Callback CurrentMeasurement: powericon('ThreePhaseVIMeasurementCback',gcb,'');
      mask Callback SetLabelI: powericon('ThreePhaseVIMeasurementCback',gcb,'');
      mask Callback LabelI: powericon('ThreePhaseVIMeasurementCback',gcb,'');
      mask Callback Ipu: powericon('ThreePhaseVIMeasurementCback',gcb,'');
      mask TypeOptions OutputType: Complex | Real-Imag | Magnitude-Angle | Magnitude
  Bus_Fault : powerlib/Measurements/Three-Phase V-I Measurement  VoltageMeasurement=no  SetLabelV=on  LabelV=Test_Parallel_V  Vpu=off  VpuLL=off  CurrentMeasurement=yes  SetLabelI=off  LabelI=Fault_Iabc  Ipu=off  Pbase=Pnom  Vbase=Vac  OutputType=Complex  PhasorSimulation=off  PSBequivalent=0
  CT-ratio : Gain  Gain=1/100  SaturateOnIntegerOverflow=on  OutDataTypeStr=Inherit: Same as input  ParamDataTypeStr=Inherit: Same as input
  CT-ratio1 : Gain  Gain=1/100  SaturateOnIntegerOverflow=on  OutDataTypeStr=Inherit: Same as input  ParamDataTypeStr=Inherit: Same as input
  CT-ratio2 : Gain  Gain=1/100  SaturateOnIntegerOverflow=on  OutDataTypeStr=Inherit: Same as input  ParamDataTypeStr=Inherit: Same as input
  Constant3 : Constant
  Controllable Fault : Subsystem  Commented=on  mask{Fault_Start_Time=1, Fault_Base_Duration_time=0.2, Fault_Ramp_End_Time=2, Fault_Base_Voltage_pu=0.6, Fault_End_Voltage_pu=1}
      mask prompts: Fault_Start_Time "Set fault start time (s)"; Fault_Base_Duration_time "Set base fault duration (Δs)"; Fault_Ramp_End_Time "Set fault ramp end time (s)"; Fault_Base_Voltage_pu "Set base voltage amplitude (p.u.)"; Fault_End_Voltage_pu "Set end voltage amplitude (p.u.)"
      mask init:
      | % % Fault base voltage V calculation
      | 
      | % Fault ramp rate pu/s calculation
      | x1=Fault_Start_Time + Fault_Base_Duration_time;
      | y1=Fault_Base_Voltage_pu;
      | x2=Fault_Ramp_End_Time;
      | y2=Fault_End_Voltage_pu;
      | Fault_Ramp_Rate=(y2-y1)/(x2-x1);
      | Fault_Ramp_Rate_VoltageSourceBlock= (y2/y1-1)/(x2-x1);
      | 
      | Simulation_Time= str2num(get_param(bdroot, 'StopTime'));
      mask DialogControl Container1 Prompt: Time variables
      mask DialogControl Container2 Prompt: Voltage variables
      mask Display: image('Fault2.png')
  Differential Element 1 : Subsystem  Commented=on  mask{Freq=50, bias=[ 0 200;10000 5000], Cpg=2.2660e-07, Cpp=2E-9, CT_local=100, CT_remote=100, PT_local=2000, CT_local_dir=1, CT_remote_dir=-1}
      mask prompts: Freq "Fundamental Frequency (Hz):"; bias "Bias Characteristic [A], e.g.  [R1, D1; R2, D2]"; Cpg "Capacitance between phase and ground (F)"; Cpp "Mutual Capacitance between phases (F)"; CT_local "CT ratio local"; CT_remote "CT ratio remote"; PT_local "PT ratio local"; CT_local_dir "local CT direction (positive = 1; negative = -1)"; CT_remote_dir "remote CT direction (positive = 1; negative = -1)"
      mask DialogControl DescTextVar Prompt: This protection block expects secondary input values.
      mask DialogControl Container14 Prompt: General
      mask DialogControl Container8 Prompt: The bias Characteristic is to be defined by primary values.
      mask DialogControl ParameterGroupVar Prompt: Charging current compensation
      mask DialogControl Container13 Prompt: Voltage and current transformers
      mask DialogControl ParameterCTChar Prompt: Positive current direction is towards the protected element
  Differential Element 2 : Subsystem  Commented=on  mask{Freq=50, bias=[ 0 200;10000 5000], Cpg=2.2660e-07, Cpp=2E-9, CT_local=100, CT_remote=100, PT_local=2000, CT_local_dir=1, CT_remote_dir=-1}
      mask prompts: Freq "Fundamental Frequency (Hz):"; bias "Bias Characteristic [A], e.g.  [R1, D1; R2, D2]"; Cpg "Capacitance between phase and ground (F)"; Cpp "Mutual Capacitance between phases (F)"; CT_local "CT ratio local"; CT_remote "CT ratio remote"; PT_local "PT ratio local"; CT_local_dir "local CT direction (positive = 1; negative = -1)"; CT_remote_dir "remote CT direction (positive = 1; negative = -1)"
      mask DialogControl DescTextVar Prompt: This protection block expects secondary input values.
      mask DialogControl Container14 Prompt: General
      mask DialogControl Container8 Prompt: The bias Characteristic is to be defined by primary values.
      mask DialogControl ParameterGroupVar Prompt: Charging current compensation
      mask DialogControl Container13 Prompt: Voltage and current transformers
      mask DialogControl ParameterCTChar Prompt: Positive current direction is towards the protected element
  "Dummy Bus Signals " : Subsystem
  Dummy WF signals : Subsystem
  Fault_timing_generator : Subsystem
  From{10,49..53,58,66} (8 alike) : From  Commented=on  GotoTag=EnableProtection
  From11 : From  Commented=on  GotoTag=V_2
  From{17,30..31,33,42} (5 alike) : From  Commented=on  GotoTag=I_2
  From{9,18..19,38,47,63} (6 alike) : From  Commented=on  GotoTag=I_1
  From3 : From  Commented=on  GotoTag=wind
  From32 : From  Commented=on  GotoTag=I_3
  From34 : From  Commented=on  GotoTag=V_2
  From35 : From  Commented=on  GotoTag=Trip_OC_1
  From36 : From  Commented=on  GotoTag=Trip_Diff_1
  From37 : From  Commented=on  GotoTag=Trip_Z_1
  From39 : From  Commented=on  GotoTag=V_1
  From40 : From  Commented=on  GotoTag=V_2
  From43 : From  Commented=on  GotoTag=Trip_TF_diff
  From44 : From  Commented=on  GotoTag=Trip_OC_2
  From45 : From  Commented=on  GotoTag=Trip_Diff_2
  From46 : From  Commented=on  GotoTag=Trip_Z_2
  From48 : From  Commented=on  GotoTag=V_1
  From54 : From  Commented=on  GotoTag=I_4
  From55 : From  Commented=on  GotoTag=I_3
  From56 : From  Commented=on  GotoTag=V_3
  From57 : From  Commented=on  GotoTag=V_4
  From59 : From  Commented=on  GotoTag=V_1
  From60 : From  Commented=on  GotoTag=Trip_1
  From61 : From  Commented=on  GotoTag=Trip_2
  From62 : From  Commented=on  GotoTag=Trip_3
  From64 : From  Commented=on  GotoTag=Trip_IN_OC_1
  From8 : From  Commented=on  GotoTag=I_4
  Goto23 : Goto  Commented=on  GotoTag=Trip_Diff_2
  Goto24 : Goto  Commented=on  GotoTag=Trip_Z_2
  Goto25 : Goto  Commented=on  GotoTag=Trip_TF_diff
  Goto26 : Goto  Commented=on  GotoTag=Trip_Diff_1
  Goto27 : Goto  Commented=on  GotoTag=Trip_Z_1
  Goto33 : Goto  Commented=on  GotoTag=EnableProtection
  Goto35 : Goto  Commented=on  GotoTag=Trip_1
  Goto36 : Goto  Commented=on  GotoTag=Trip
  Goto37 : Goto  Commented=on  GotoTag=Trip_3
  Goto39 : Goto  Commented=on  GotoTag=Trip_2
  Goto40 : Goto  Commented=on  GotoTag=Trip_IN_OC_1
  Goto6 : Goto  Commented=on  GotoTag=Trip_OC_1
  Goto7 : Goto  Commented=on  GotoTag=Trip_OC_2
  Ground1 : powerlib/Elements/Ground  LConnTagsString=a
  Ground2 : powerlib/Elements/Ground  LConnTagsString=a
  Impedance Element 1 : Subsystem  Commented=on  mask(Distance Relay Settings:){ZoneImpedance=[1.04 2.03 0.52 3.5], ZoneTime=[0 0.33 1 0.66], LineAngle=84.0, k0m1=0.726, k0a1=-3.69, underV=110*0.8, Freq=50}
      mask prompts: ZoneImpedance "Zone impedances [Z1  Z2  Z3  Z4] (Ohm):"; ZoneTime "Zone times [T1  T2  T3  T4] (s):"; LineAngle "Line angle (deg):"; underV "UnderVoltage Threshold (V):"; Freq "Fundamental frequency (Hz):"
      mask DialogControl DescTextVar Prompt: Distance element: Mho-relay. Siemens relays in lab have quadrilateral zones.
  Impedance Element 2 : Subsystem  Commented=on  mask(Distance Relay Settings:){ZoneImpedance=[1.04 2.03 0.52 3.5], ZoneTime=[0 0.33 1 0.66], LineAngle=84.0, k0m1=0.726, k0a1=-3.69, underV=110*0.8, Freq=50}
      mask prompts: ZoneImpedance "Zone impedances [Z1  Z2  Z3  Z4] (Ohm):"; ZoneTime "Zone times [T1  T2  T3  T4] (s):"; LineAngle "Line angle (deg):"; underV "UnderVoltage Threshold (V):"; Freq "Fundamental frequency (Hz):"
      mask DialogControl DescTextVar Prompt: Distance element: Mho-relay. Siemens relays in lab have quadrilateral zones.
  Multiport Switch : MultiPortSwitch  Inputs=10  DiagnosticForDefault=Warning  InputSameDT=on
  Multiport Switch1 : MultiPortSwitch  Inputs=4  DiagnosticForDefault=Warning  InputSameDT=on
      settings: LockScale=on
  OR : Logic  Commented=on  Operator=OR  Inputs=3  IconShape=distinctive  AllPortsSameDT=off  OutDataTypeStr=boolean
  Overcurrent Element 1 : Subsystem  Commented=on  mask(Overcurrent Relay){Iop=12, Td=0.2, ResCurr=0.1, Freq=50}
      mask prompts: Iop "Pickup Current (A - peak):"; Td "Time Delay (s):"; ResCurr "Zero Sequence Current Component Threshold (A - peak):"; Freq "Fundamental Frequency (Hz):"
  Overcurrent Element 2 : Subsystem  Commented=on  mask(Overcurrent Relay){Iop=6, Td=0.2, ResCurr=0.1, Freq=50}
      mask prompts: Iop "Pickup Current (A - peak):"; Td "Time Delay (s):"; ResCurr "Zero Sequence Current Component Threshold (A - peak):"; Freq "Fundamental Frequency (Hz):"
  Overcurrent Inverse time : Subsystem  Commented=on  mask(Overcurrent Relay){Freq=50, TMS=1, CtrlSig=3, Iop=15}
      mask prompts: Freq "Fundamental Frequency (Hz):"; TMS "Time Multiplier Setting (TMS)"; CtrlSig "Type of curve (1 = inverse; 2=Very inverse; 3=Extremely inverse)"; Iop "Pickup Setting (A)"
      mask DialogControl DescTextVar Prompt: Inverse time characteristics of Overcurrent Relay based on IEC 60255
  Qref_pu{1,3,11,14,24,33} (6 alike) : Constant  Value=0
  Qref_pu2 : Constant  Commented=on  Value=0
  Scope Bus{1..4} (4 alike) : Scope  Commented=on  NumInputPorts=3
  Scope{1..17} (17 alike) : Scope  NumInputPorts=3
  Step : Step  Commented=on  Time=0.5
  Subsystem1 : Subsystem
  Subsystem10 : Subsystem
  Subsystem11 : Subsystem
  Subsystem12 : Subsystem
  Subsystem13 : Subsystem
  Subsystem14 : Subsystem
  Subsystem15 : Subsystem
  Subsystem16 : Subsystem
  Subsystem17 : Subsystem
  Subsystem18 : Subsystem
  Subsystem19 : Subsystem
  Subsystem2 : Subsystem
  Subsystem3 : Subsystem  Commented=on
  Subsystem4 : Subsystem  Commented=on
  Subsystem5 : Subsystem
  Subsystem6 : Subsystem
  Subsystem7 : Subsystem
  Subsystem8 : Subsystem
  Subsystem9 : Subsystem
  Terminator1 : Terminator
  Three-Phase Breaker {,1..19,22..23,25..29,38..39,41} (30 alike) : powerlib/Elements/Three-Phase Breaker  InitialState=closed  SwitchA=on  SwitchB=on  SwitchC=on  SwitchTimes=100  External=off  BreakerResistance=0.01  SnubberResistance=1e6  SnubberCapacitance=1e-10  Measurements=None
  Three-Phase Fault : powerlib/Elements/Three-Phase Fault  InitialStates=0  FaultA=on  FaultB=off  FaultC=on  GroundFault=on  SwitchTimes="[1  2]"  External=on  SwitchStatus=NaN  FaultResistance=0.01  GroundResistance=0.01  SnubberResistance=1e6  SnubberCapacitance=inf  Measurements=None
  Transformer differential element 1 : Subsystem  Commented=on  mask{Parameter1=50}
      mask prompts: Parameter1 "Fundamental frequency (Hz):"
      mask DialogControl DescTextVar Prompt: Please adjust the parameters in the two blocks below to configure your protection settings.
  Unit Delay : UnitDelay  SampleTime=Ts_Power  HasFrameUpgradeWarning=on
  VT-ratio : Gain  Gain=1/2000  SaturateOnIntegerOverflow=on  OutDataTypeStr=Inherit: Same as input  ParamDataTypeStr=Inherit: Same as input
  VT-ratio1 : Gain  Gain=1/2000  SaturateOnIntegerOverflow=on  OutDataTypeStr=Inherit: Same as input  ParamDataTypeStr=Inherit: Same as input
  VT-ratio2 : Gain  Gain=1/2000  SaturateOnIntegerOverflow=on  OutDataTypeStr=Inherit: Same as input  ParamDataTypeStr=Inherit: Same as input
  Vac kV1 : powerlib/Electrical Sources/Three-Phase Programmable Voltage Source  PositiveSequence=[Vac 0 freq]  VariationEntity=None  VariationType=Table of time-amplitude pairs  VariationTypeAlt=Step  VariationStep=-0.2  VariationRate=10  VariationMagnitude=0.3  VariationFrequency=60  VariationTiming=[0.05 0.05+5/60]  VariationPhaseA=off  Amplitudes=[1 0.75 1.0]  TimeValues=[0 0.03 0.13]  HarmonicGeneration=off  HarmonicA=[1 -0.1 0 2]  HarmonicB=[2 0.15 35 2]*0  Timing="[0.1  2]"  BusType=swing  Pref=0  Qref=0  Qmin=-inf  Qmax=inf
  Vac kV2 : powerlib/Electrical Sources/Three-Phase Programmable Voltage Source  PositiveSequence=[Vac 0 freq]  VariationEntity=None  VariationType=Table of time-amplitude pairs  VariationTypeAlt=Step  VariationStep=-0.2  VariationRate=10  VariationMagnitude=0.3  VariationFrequency=60  VariationTiming=[0.05 0.05+5/60]  VariationPhaseA=off  Amplitudes=[1 0.75 1.0]  TimeValues=[0 0.03 0.13]  HarmonicGeneration=off  HarmonicA=[1 -0.1 0 2]  HarmonicB=[2 0.15 35 2]*0  Timing="[0.1  2]"  BusType=swing  Pref=0  Qref=0  Qmin=-inf  Qmax=inf
  Wind Type IV Detailed v2.1 - 1 : Subsystem  LoadFcn=%find_system(gcs,'FollowLinks', 'on', 'LookUnderMasks', 'all');  mask(Wind Turbine: Model 7){Nb_wt=10, Pnom=15e6, Vgrid=66000, CutIn_Wind_Speed=3, Rated_Wind_Speed=12, CutOut_Wind_Speed=25, Power_Data_Filled=No, Title=Power Data (W), Wind_Characteristics1=0, Wind_Characteristics2=0, Wind_Characteristics3=0, Wind_Characteristics4=0, Wind_Characteristics5=0, Wind_Characteristics6=0.1e6, Wind_Characteristics7=0.2e6, Wind_Characteristics8=0.3e6, Wind_Characteristics9=0.4e6, Wind_Characteristics10=0.5e6, Wind_Characteristics11=0.6e6, Wind_Characteristics12=0.7e6, Wind_Characteristics13=0.8e6, Wind_Characteristics14=0.9e6, Wind_Characteristics15=1, Wind_Characteristics16=1, Wind_Characteristics17=1, Wind_Characteristics18=1, Wind_Characteristics19=1, Wind_Characteristics20=1, Wind_Characteristics21=1, Wind_Characteristics22=1, Wind_Characteristics23=1, Wind_Characteristics24=1, Wind_Characteristics25=1, Wind_Characteristics26=[], Wind_Characteristics27=[], Wind_Characteristics28=[], Wind_Characteristics29=[], Wind_Characteristics30=[], Wind_Characteristics31=[], Wind_Characteristics32=[], Wind_Characteristics33=[], Wind_Characteristics34=[], Wind_Characteristics35=[], Power_Curve_Export=No, Visualization_save_PowerGraph_path='', Fault_Base_Duration_time_FRT=0.2, Fault_Ramp_End_Time_FRT=0.1, Fault_Base_Voltage_pu_FRT=0.1, Fault_End_Voltage_pu_FRT=0.85, FRT_Graph_Export=No, Visualization_save_FRT_path='', Ts=Ts}
      mask prompts: Nb_wt "Number of wind turbines [Nb_wt]"; Pnom "Wind turbine nominal power (W) [Pnom]"; Vgrid "Grid Voltage RMS (line-line) (V) [Vgrid]"; CutIn_Wind_Speed "Cut-in Wind Speed (m/s)"; Rated_Wind_Speed "Rated Wind Speed (m/s)"; CutOut_Wind_Speed "Cut-out Wind Speed (m/s)"; Power_Data_Filled "Was Power vs. Wind speed data obtained?"; Title "Wind Speed (m/s)"; Wind_Characteristics1 "1"; Wind_Characteristics2 "2"; Wind_Characteristics3 "3"; Wind_Characteristics4 "4"; Wind_Characteristics5 "5"; Wind_Characteristics6 "6"; Wind_Characteristics7 "7"; Wind_Characteristics8 "8"; Wind_Characteristics9 "9"; Wind_Characteristics10 "10"; Wind_Characteristics11 "11"; Wind_Characteristics12 "12"; Wind_Characteristics13 "13"; Wind_Characteristics14 "14"; Wind_Characteristics15 "15"; Wind_Characteristics16 "16"; Wind_Characteristics17 "17"; Wind_Characteristics18 "18"; Wind_Characteristics19 "19"; Wind_Characteristics20 "20"; Wind_Characteristics21 "21"; Wind_Characteristics22 "22"; Wind_Characteristics23 "23"; Wind_Characteristics24 "24"; Wind_Characteristics25 "25"; Wind_Characteristics26 "26"; Wind_Characteristics27 "27"; Wind_Characteristics28 "28"; Wind_Characteristics29 "29"; Wind_Characteristics30 "30"; Wind_Characteristics31 "31"; Wind_Characteristics32 "32"; Wind_Characteristics33 "33"; Wind_Characteristics34 "34"; Wind_Characteristics35 "35"; Power_Curve_Export "Export Power vs. Wind speed curve?"; Visualization_save_PowerGraph_path "Enter file path for the figures"; Fault_Base_Duration_time_FRT "Set base fault duration (Δs)"; Fault_Ramp_End_Time_FRT "Set post-fault ramp duration (Δs)"; Fault_Base_Voltage_pu_FRT "Set base voltage amplitude (p.u.)"; Fault_End_Voltage_pu_FRT "Set end voltage amplitude (p.u.)"; FRT_Graph_Export "Export FRT Code graph?"; Visualization_save_FRT_path "Enter file path for the figures"
      mask help: This block implements a model of a variable speed pitch controlled wind turbine using a synchronous generator.
      mask init:
      | Q_nom_grid=Pnom*0.2;
      | % Fnom=50;
      | 
      | Vnom=690;
      | Vnom_gen=Vnom;
      | Inom=Pnom/Vnom_gen;
      | 
      | % Converter
      | C_DClink=1800e-3;
      | Vdc_nom=1100;
      | Q_filter=50;
      | 
      | % Controller data
      | Freq_filter=10000;   %Hz
      | Zeta_filter=0.707;
      | 
      | Freq_sawtooth=2000; %Hz, Boost converter
      | Freq_PWM=3000; %Hz, Inverter
      | 
      | % Turbine data
      | % Wind turbine:
      | R_turb = 42; % [m]
      | ro_air = 1.225; % air density
      | vspeed_max = 11; % [m/s]
      | vspeed_min = 4; % [m/s]
      | lambda_opt = 7.1;
      | w_init = 1.878; % [rad/s]
      | wr_ref_tau = 8; % [s]
      | 
      | C_var_filter=150e3;
      | 
      | 
      | %{ 
      | Create power curve
      | %}
      | 
      | v_wind_table = 1:1:35;
      | 
      | %% All variables imported and converted to doubles to avoid errors
      | CutIn_Wind_Speed=ceil(str2double(get_param(gcb,'CutIn_Wind_Speed')));                                                       % Cut-in speed (m/s)
      | CutOut_Wind_Speed=ceil(str2double(get_param(gcb,'CutOut_Wind_Speed')));                                                     % Cut-out speed (m/s)
      | Rated_Wind_Speed=ceil(str2double(get_param(gcb,'Rated_Wind_Speed')));                                                       % Rated speed (m/s)
      | Power_Data_Filled=get_param(gcb,'Power_Data_Filled');
      | v_input = v_wind_table;
      | n_rows=size(v_wind_table,2);
      | v_in_matrix=zeros (1,n_rows) + CutIn_Wind_Speed;                                                                            % Convert input values to usable arrays
      | v_out_matrix=zeros (1,n_rows) + CutOut_Wind_Speed;
      | v_rated_matrix=zeros (1,n_rows) + Rated_Wind_Speed;
      | %% Create power data table
      | if Power_Data_Filled == "Yes"                                                                                               %The input data will be smoothened out        
      |     powervbins=zeros(1,35);
      |     for i = 1:35
      |         index=sprintf('%.0f',i);
      |         wind_characteristics_indexed=strcat('Wind_Characteristics',index);
      |         powervbins(1,i)=str2double(get_param(gcb,wind_characteristics_indexed));
      |     end  
      |     for i= round(CutIn_Wind_Speed):round(Rated_Wind_Speed) 
      |         if isnan( powervbins(1,i))
      |             powervbins(1,i) = ((v_input(1 , i)^2 - CutIn_Wind_Speed^2)./(Rated_Wind_Speed^2 - CutIn_Wind_Speed^2))*Pnom;
      |         else      
      |         end  
      |     end
      |     powervbins(v_input < v_in_matrix ) = 0;
      |     powervbins(v_input > v_out_matrix ) = 0;
      |     powervbins(v_input >= Rated_Wind_Speed & v_input <= CutOut_Wind_Speed ) = Pnom;
      |     Curated_Wind_Power_Data=powervbins;  
      | else                                                                                                                        %Default P vs v_wind will be applied
      |     powervbins = ((v_input.^2 - v_in_matrix.^2)./(v_rated_matrix.^2 - v_in_matrix.^2)).*Pnom;                               % Calculating power curve
      |     powervbins(v_input < v_in_matrix) = 0;                                                                                  %Care, using this formula P=0 at v_in
      |     powervbins(v_input > v_out_matrix) = 0;
      |     powervbins(v_input >= Rated_Wind_Speed & v_input <= CutOut_Wind_Speed) = Pnom;
      |     Curated_Wind_Power_Data=powervbins;    
      | end
      | 
      | %% Plot power curve
      | trigger_power_graph=get_param(gcb,'Power_Curve_Export');%%%%%%%%%%%%%%%%%%%%%%%%%%%                                                                                                                   
      | if strcmp(trigger_power_graph,"Print") || strcmp(trigger_power_graph,"Print and save")
      |     fontsize=20;
      |     figure; plot(1:1:35,Curated_Wind_Power_Data/Pnom,'b', 'LineWidth', 2);
      |     xlabel('Velocity (m/s)','FontSize', fontsize-5);
      |     ylabel('Turbine power (p.u.)','FontSize', fontsize-5);
      |     title('Wind Turbine Power Curve','FontSize', fontsize-1);
      |     offset = 0.1;
      |     for i=1:length(powervbins)
      |         if not (Curated_Wind_Power_Data(i)/Pnom== 0) & not (powervbins(i)/Pnom== 1)
      |             text(i+.1,Curated_Wind_Power_Data(i)/Pnom,['(' num2str(i),' m/s; ' num2str(Curated_Wind_Power_Data(i)/Pnom) ' p.u.)']);
      |         end
      |     end
      |     text(Rated_Wind_Speed+.1,Curated_Wind_Power_Data(round(Rated_Wind_Speed))/Pnom-.02,['v_r_a_t_e_d (' num2str(Rated_Wind_Speed),' m/s; ' num2str(Curated_Wind_Power_Data(round(Rated_Wind_Speed))/Pnom) ' p.u.)']);
      |     text(CutOut_Wind_Speed+.1,Curated_Wind_Power_Data(round(CutOut_Wind_Speed))/Pnom-.02,['v_o_u_t (' num2str(CutOut_Wind_Speed),' m/s; ' num2str(Curated_Wind_Power_Data(round(CutOut_Wind_Speed))/Pnom) ' p.u.)']);
      | end
      | %% Saving power curve as .fig
      | if strcmp(trigger_power_graph,"Print and save")
      |     file_name='Wind turbine power curve';
      |     saveas(gca, fullfile(Visualization_save_PowerGraph_path, file_name), 'fig');
      | end
      | 
      | 
      | %%%% Fault Ride Through Characteristic %%%%
      | 
      | %% Get values from 'Grid Code FRT' mask in the model
      | Fault_Start_Time_FRT=1;%str2double(get_param(gcb,'Fault_Start_Time_FRT'));
      | Fault_Base_Duration_time_FRT=str2double(get_param(gcb,'Fault_Base_Duration_time_FRT'));
      | Fault_Ramp_End_Time_FRT=Fault_Start_Time_FRT+Fault_Base_Duration_time_FRT+str2double(get_param(gcb,'Fault_Ramp_End_Time_FRT'));
      | Fault_Base_Voltage_pu_FRT=str2double(get_param(gcb,'Fault_Base_Voltage_pu_FRT'));
      | Fault_End_Voltage_pu_FRT=str2double(get_param(gcb,'Fault_End_Voltage_pu_FRT'));
      | % Ts is in the base workspace already
      | % Simulation_Time= str2double(get_param(gcs, 'StopTime'));
      | Simulation_Time=3;%%Dirty Patch to make RT work
      | %% Ramp rate calculation
      | x1=Fault_Start_Time_FRT + Fault_Base_Duration_time_FRT;
      | y1=Fault_Base_Voltage_pu_FRT;
      | x2=Fault_Ramp_End_Time_FRT;
      | y2=Fault_End_Voltage_pu_FRT;
      | Fault_Ramp_Rate_FRT = ((y2 - y1) / (x2 - x1));
      | %% Generate Grid Code graph
      | time_interval=Ts;
      | j=0;
      | len=Simulation_Time/Ts+1;
      | Grid_Code_Timetable_FRT = zeros(len,2);
      | for i=1:length(0:time_interval:Fault_Start_Time_FRT)
      |     Grid_Code_Timetable_FRT (i,1)=[j];
      |     Grid_Code_Timetable_FRT (i,2)=[1];
      |     j=j+time_interval;
      | end
      | i=i+1;
      | for i=i:i+length(Fault_Start_Time_FRT:time_interval:Fault_Start_Time_FRT+Fault_Base_Duration_time_FRT)-1
      |     Grid_Code_Timetable_FRT (i,1)=[j];
      |     Grid_Code_Timetable_FRT (i,2)=[Fault_Base_Voltage_pu_FRT];
      |     j=j+time_interval;
      | end
      | % Conversion of ramp_rate from pu/s to pu/time_interval
      | Fault_Ramp_Rate_Adjusted_FRT=Fault_Ramp_Rate_FRT*time_interval;
      | j=j-time_interval;
      | for i=i:i+length(Fault_Start_Time_FRT+Fault_Base_Duration_time_FRT:time_interval:Fault_Ramp_End_Time_FRT)-1
      |     Grid_Code_Timetable_FRT (i,1)=[j];
      |     Grid_Code_Timetable_FRT(i,2)=[Grid_Code_Timetable_FRT(i-1,2)+Fault_Ramp_Rate_Adjusted_FRT];
      |     j=j+time_interval;
      | end
      | j=j-time_interval;
      | for i=i:i+length(Fault_Ramp_End_Time_FRT:time_interval:Simulation_Time)-2
      |     Grid_Code_Timetable_FRT (i,1)=[j];
      |     Grid_Code_Timetable_FRT(i,2)=[Fault_End_Voltage_pu_FRT];
      |     j=j+time_interval;
      | end
      | 
      | %% Print Function
      | % Print
      | trigger_FRT_graph=get_param(gcb,'FRT_Graph_Export');
      | if strcmp(trigger_FRT_graph,"Print") || strcmp(trigger_FRT_graph,"Print and save")
      |     fontsize=20;
      |     figure
      |     plot(Grid_Code_Timetable_FRT(:,1),Grid_Code_Timetable_FRT(:,2),'b', 'LineWidth', 2);
      |     set(gca,'YLim',[0 1.5])
      |     set(gca,'YTick',(0:0.1:1.5))
      |     set(gca,'XTick',(0:0.1:4))
      |     xlabel('Time (s)','FontSize', fontsize-5);
      |     ylabel('Grid voltage (p.u.)','FontSize', fontsize-5);
      |     title('Grid fault characteristics','FontSize', fontsize-1);
      |     offset = 0.1;
      | end
      | % Saving FRT graph as .fig
      | if strcmp(trigger_FRT_graph,"Print and save")
      |     file_name='FRT grid code requirement graph';
      |     saveas(gca, fullfile(Visualization_save_FRT_path, file_name), 'fig');
      | end
      mask TypeOptions CutIn_Wind_Speed: 1 | 2 | 3 | 4 | 5 | 6 | 7 | 8 | 9 | 10 | 11 | 12 | 13 | 14 | 15 | 16 | 17 | 18 | 19 | 20 | 21 | 22 | 23 | 24 | 25 | 26 | 27 | 28 | 29 | 30 | 31 | 32 | 33 | 34 | 35
      mask TypeOptions Rated_Wind_Speed: 1 | 2 | 3 | 4 | 5 | 6 | 7 | 8 | 9 | 10 | 11 | 12 | 13 | 14 | 15 | 16 | 17 | 18 | 19 | 20 | 21 | 22 | 23 | 24 | 25 | 26 | 27 | 28 | 29 | 30 | 31 | 32 | 33 | 34 | 35
      mask TypeOptions CutOut_Wind_Speed: 1 | 2 | 3 | 4 | 5 | 6 | 7 | 8 | 9 | 10 | 11 | 12 | 13 | 14 | 15 | 16 | 17 | 18 | 19 | 20 | 21 | 22 | 23 | 24 | 25 | 26 | 27 | 28 | 29 | 30 | 31 | 32 | 33 | 34 | 35
      mask TypeOptions Power_Data_Filled: Yes | No
      mask TypeOptions Power_Curve_Export: Print | Print and save | No
      mask TypeOptions FRT_Graph_Export: Print | Print and save | No
      mask DialogControl Container8 Prompt: General data
      mask DialogControl Container11 Prompt: Power data per turbine
      mask DialogControl Control2 Prompt: If no wind speed characteristics were found for the turbine the variables below may be set at their default values.
      mask DialogControl Power_Data_Table Prompt: If data for a certain wind speed is not found leave blank ([]). Power >= v_out and <=v_in shall not be filled.
      mask DialogControl Container16 Prompt: Fault ride through settings
      mask DialogControl Container17 Prompt: Time variables
      mask DialogControl Container18 Prompt: Voltage thresholds
      mask Display: image('windturbine4.jpg')
  Wind Type IV Detailed v2.1 - 11 : Subsystem  LoadFcn=%find_system(gcs,'FollowLinks', 'on', 'LookUnderMasks', 'all');  mask(Wind Turbine: Model 7){Nb_wt=24, Pnom=15e6, Vgrid=66000, CutIn_Wind_Speed=3, Rated_Wind_Speed=12, CutOut_Wind_Speed=25, Power_Data_Filled=No, Title=Power Data (W), Wind_Characteristics1=0, Wind_Characteristics2=0, Wind_Characteristics3=0, Wind_Characteristics4=0, Wind_Characteristics5=0, Wind_Characteristics6=0.1e6, Wind_Characteristics7=0.2e6, Wind_Characteristics8=0.3e6, Wind_Characteristics9=0.4e6, Wind_Characteristics10=0.5e6, Wind_Characteristics11=0.6e6, Wind_Characteristics12=0.7e6, Wind_Characteristics13=0.8e6, Wind_Characteristics14=0.9e6, Wind_Characteristics15=1, Wind_Characteristics16=1, Wind_Characteristics17=1, Wind_Characteristics18=1, Wind_Characteristics19=1, Wind_Characteristics20=1, Wind_Characteristics21=1, Wind_Characteristics22=1, Wind_Characteristics23=1, Wind_Characteristics24=1, Wind_Characteristics25=1, Wind_Characteristics26=[], Wind_Characteristics27=[], Wind_Characteristics28=[], Wind_Characteristics29=[], Wind_Characteristics30=[], Wind_Characteristics31=[], Wind_Characteristics32=[], Wind_Characteristics33=[], Wind_Characteristics34=[], Wind_Characteristics35=[], Power_Curve_Export=No, Visualization_save_PowerGraph_path='', Fault_Base_Duration_time_FRT=0.2, Fault_Ramp_End_Time_FRT=0.1, Fault_Base_Voltage_pu_FRT=0.1, Fault_End_Voltage_pu_FRT=0.85, FRT_Graph_Export=No, Visualization_save_FRT_path='', Ts=Ts}
      mask prompts: Nb_wt "Number of wind turbines [Nb_wt]"; Pnom "Wind turbine nominal power (W) [Pnom]"; Vgrid "Grid Voltage RMS (line-line) (V) [Vgrid]"; CutIn_Wind_Speed "Cut-in Wind Speed (m/s)"; Rated_Wind_Speed "Rated Wind Speed (m/s)"; CutOut_Wind_Speed "Cut-out Wind Speed (m/s)"; Power_Data_Filled "Was Power vs. Wind speed data obtained?"; Title "Wind Speed (m/s)"; Wind_Characteristics1 "1"; Wind_Characteristics2 "2"; Wind_Characteristics3 "3"; Wind_Characteristics4 "4"; Wind_Characteristics5 "5"; Wind_Characteristics6 "6"; Wind_Characteristics7 "7"; Wind_Characteristics8 "8"; Wind_Characteristics9 "9"; Wind_Characteristics10 "10"; Wind_Characteristics11 "11"; Wind_Characteristics12 "12"; Wind_Characteristics13 "13"; Wind_Characteristics14 "14"; Wind_Characteristics15 "15"; Wind_Characteristics16 "16"; Wind_Characteristics17 "17"; Wind_Characteristics18 "18"; Wind_Characteristics19 "19"; Wind_Characteristics20 "20"; Wind_Characteristics21 "21"; Wind_Characteristics22 "22"; Wind_Characteristics23 "23"; Wind_Characteristics24 "24"; Wind_Characteristics25 "25"; Wind_Characteristics26 "26"; Wind_Characteristics27 "27"; Wind_Characteristics28 "28"; Wind_Characteristics29 "29"; Wind_Characteristics30 "30"; Wind_Characteristics31 "31"; Wind_Characteristics32 "32"; Wind_Characteristics33 "33"; Wind_Characteristics34 "34"; Wind_Characteristics35 "35"; Power_Curve_Export "Export Power vs. Wind speed curve?"; Visualization_save_PowerGraph_path "Enter file path for the figures"; Fault_Base_Duration_time_FRT "Set base fault duration (Δs)"; Fault_Ramp_End_Time_FRT "Set post-fault ramp duration (Δs)"; Fault_Base_Voltage_pu_FRT "Set base voltage amplitude (p.u.)"; Fault_End_Voltage_pu_FRT "Set end voltage amplitude (p.u.)"; FRT_Graph_Export "Export FRT Code graph?"; Visualization_save_FRT_path "Enter file path for the figures"
      mask help: This block implements a model of a variable speed pitch controlled wind turbine using a synchronous generator.
      mask init: same as Versie2/SM_WT1/Wind Type IV Detailed v2.1 - 1
      mask TypeOptions CutIn_Wind_Speed: 1 | 2 | 3 | 4 | 5 | 6 | 7 | 8 | 9 | 10 | 11 | 12 | 13 | 14 | 15 | 16 | 17 | 18 | 19 | 20 | 21 | 22 | 23 | 24 | 25 | 26 | 27 | 28 | 29 | 30 | 31 | 32 | 33 | 34 | 35
      mask TypeOptions Rated_Wind_Speed: 1 | 2 | 3 | 4 | 5 | 6 | 7 | 8 | 9 | 10 | 11 | 12 | 13 | 14 | 15 | 16 | 17 | 18 | 19 | 20 | 21 | 22 | 23 | 24 | 25 | 26 | 27 | 28 | 29 | 30 | 31 | 32 | 33 | 34 | 35
      mask TypeOptions CutOut_Wind_Speed: 1 | 2 | 3 | 4 | 5 | 6 | 7 | 8 | 9 | 10 | 11 | 12 | 13 | 14 | 15 | 16 | 17 | 18 | 19 | 20 | 21 | 22 | 23 | 24 | 25 | 26 | 27 | 28 | 29 | 30 | 31 | 32 | 33 | 34 | 35
      mask TypeOptions Power_Data_Filled: Yes | No
      mask TypeOptions Power_Curve_Export: Print | Print and save | No
      mask TypeOptions FRT_Graph_Export: Print | Print and save | No
      mask DialogControl Container8 Prompt: General data
      mask DialogControl Container11 Prompt: Power data per turbine
      mask DialogControl Control2 Prompt: If no wind speed characteristics were found for the turbine the variables below may be set at their default values.
      mask DialogControl Power_Data_Table Prompt: If data for a certain wind speed is not found leave blank ([]). Power >= v_out and <=v_in shall not be filled.
      mask DialogControl Container16 Prompt: Fault ride through settings
      mask DialogControl Container17 Prompt: Time variables
      mask DialogControl Container18 Prompt: Voltage thresholds
      mask Display: image('windturbine4.jpg')
  Wind Type IV Detailed v2.1 - 14 : Subsystem  LoadFcn=%find_system(gcs,'FollowLinks', 'on', 'LookUnderMasks', 'all');  mask(Wind Turbine: Model 7){Nb_wt=26, Pnom=15e6, Vgrid=66000, CutIn_Wind_Speed=3, Rated_Wind_Speed=12, CutOut_Wind_Speed=25, Power_Data_Filled=No, Title=Power Data (W), Wind_Characteristics1=0, Wind_Characteristics2=0, Wind_Characteristics3=0, Wind_Characteristics4=0, Wind_Characteristics5=0, Wind_Characteristics6=0.1e6, Wind_Characteristics7=0.2e6, Wind_Characteristics8=0.3e6, Wind_Characteristics9=0.4e6, Wind_Characteristics10=0.5e6, Wind_Characteristics11=0.6e6, Wind_Characteristics12=0.7e6, Wind_Characteristics13=0.8e6, Wind_Characteristics14=0.9e6, Wind_Characteristics15=1, Wind_Characteristics16=1, Wind_Characteristics17=1, Wind_Characteristics18=1, Wind_Characteristics19=1, Wind_Characteristics20=1, Wind_Characteristics21=1, Wind_Characteristics22=1, Wind_Characteristics23=1, Wind_Characteristics24=1, Wind_Characteristics25=1, Wind_Characteristics26=[], Wind_Characteristics27=[], Wind_Characteristics28=[], Wind_Characteristics29=[], Wind_Characteristics30=[], Wind_Characteristics31=[], Wind_Characteristics32=[], Wind_Characteristics33=[], Wind_Characteristics34=[], Wind_Characteristics35=[], Power_Curve_Export=No, Visualization_save_PowerGraph_path='', Fault_Base_Duration_time_FRT=0.2, Fault_Ramp_End_Time_FRT=0.1, Fault_Base_Voltage_pu_FRT=0.1, Fault_End_Voltage_pu_FRT=0.85, FRT_Graph_Export=No, Visualization_save_FRT_path='', Ts=Ts}
      mask prompts: Nb_wt "Number of wind turbines [Nb_wt]"; Pnom "Wind turbine nominal power (W) [Pnom]"; Vgrid "Grid Voltage RMS (line-line) (V) [Vgrid]"; CutIn_Wind_Speed "Cut-in Wind Speed (m/s)"; Rated_Wind_Speed "Rated Wind Speed (m/s)"; CutOut_Wind_Speed "Cut-out Wind Speed (m/s)"; Power_Data_Filled "Was Power vs. Wind speed data obtained?"; Title "Wind Speed (m/s)"; Wind_Characteristics1 "1"; Wind_Characteristics2 "2"; Wind_Characteristics3 "3"; Wind_Characteristics4 "4"; Wind_Characteristics5 "5"; Wind_Characteristics6 "6"; Wind_Characteristics7 "7"; Wind_Characteristics8 "8"; Wind_Characteristics9 "9"; Wind_Characteristics10 "10"; Wind_Characteristics11 "11"; Wind_Characteristics12 "12"; Wind_Characteristics13 "13"; Wind_Characteristics14 "14"; Wind_Characteristics15 "15"; Wind_Characteristics16 "16"; Wind_Characteristics17 "17"; Wind_Characteristics18 "18"; Wind_Characteristics19 "19"; Wind_Characteristics20 "20"; Wind_Characteristics21 "21"; Wind_Characteristics22 "22"; Wind_Characteristics23 "23"; Wind_Characteristics24 "24"; Wind_Characteristics25 "25"; Wind_Characteristics26 "26"; Wind_Characteristics27 "27"; Wind_Characteristics28 "28"; Wind_Characteristics29 "29"; Wind_Characteristics30 "30"; Wind_Characteristics31 "31"; Wind_Characteristics32 "32"; Wind_Characteristics33 "33"; Wind_Characteristics34 "34"; Wind_Characteristics35 "35"; Power_Curve_Export "Export Power vs. Wind speed curve?"; Visualization_save_PowerGraph_path "Enter file path for the figures"; Fault_Base_Duration_time_FRT "Set base fault duration (Δs)"; Fault_Ramp_End_Time_FRT "Set post-fault ramp duration (Δs)"; Fault_Base_Voltage_pu_FRT "Set base voltage amplitude (p.u.)"; Fault_End_Voltage_pu_FRT "Set end voltage amplitude (p.u.)"; FRT_Graph_Export "Export FRT Code graph?"; Visualization_save_FRT_path "Enter file path for the figures"
      mask help: This block implements a model of a variable speed pitch controlled wind turbine using a synchronous generator.
      mask init: same as Versie2/SM_WT1/Wind Type IV Detailed v2.1 - 1
      mask TypeOptions CutIn_Wind_Speed: 1 | 2 | 3 | 4 | 5 | 6 | 7 | 8 | 9 | 10 | 11 | 12 | 13 | 14 | 15 | 16 | 17 | 18 | 19 | 20 | 21 | 22 | 23 | 24 | 25 | 26 | 27 | 28 | 29 | 30 | 31 | 32 | 33 | 34 | 35
      mask TypeOptions Rated_Wind_Speed: 1 | 2 | 3 | 4 | 5 | 6 | 7 | 8 | 9 | 10 | 11 | 12 | 13 | 14 | 15 | 16 | 17 | 18 | 19 | 20 | 21 | 22 | 23 | 24 | 25 | 26 | 27 | 28 | 29 | 30 | 31 | 32 | 33 | 34 | 35
      mask TypeOptions CutOut_Wind_Speed: 1 | 2 | 3 | 4 | 5 | 6 | 7 | 8 | 9 | 10 | 11 | 12 | 13 | 14 | 15 | 16 | 17 | 18 | 19 | 20 | 21 | 22 | 23 | 24 | 25 | 26 | 27 | 28 | 29 | 30 | 31 | 32 | 33 | 34 | 35
      mask TypeOptions Power_Data_Filled: Yes | No
      mask TypeOptions Power_Curve_Export: Print | Print and save | No
      mask TypeOptions FRT_Graph_Export: Print | Print and save | No
      mask DialogControl Container8 Prompt: General data
      mask DialogControl Container11 Prompt: Power data per turbine
      mask DialogControl Control2 Prompt: If no wind speed characteristics were found for the turbine the variables below may be set at their default values.
      mask DialogControl Power_Data_Table Prompt: If data for a certain wind speed is not found leave blank ([]). Power >= v_out and <=v_in shall not be filled.
      mask DialogControl Container16 Prompt: Fault ride through settings
      mask DialogControl Container17 Prompt: Time variables
      mask DialogControl Container18 Prompt: Voltage thresholds
      mask Display: image('windturbine4.jpg')
  Wind Type IV Detailed v2.1 - 2 : Subsystem  LoadFcn=%find_system(gcs,'FollowLinks', 'on', 'LookUnderMasks', 'all');  mask(Wind Turbine: Model 7){Nb_wt=25, Pnom=15e6, Vgrid=66000, CutIn_Wind_Speed=3, Rated_Wind_Speed=12, CutOut_Wind_Speed=25, Power_Data_Filled=No, Title=Power Data (W), Wind_Characteristics1=0, Wind_Characteristics2=0, Wind_Characteristics3=0, Wind_Characteristics4=0, Wind_Characteristics5=0, Wind_Characteristics6=0.1e6, Wind_Characteristics7=0.2e6, Wind_Characteristics8=0.3e6, Wind_Characteristics9=0.4e6, Wind_Characteristics10=0.5e6, Wind_Characteristics11=0.6e6, Wind_Characteristics12=0.7e6, Wind_Characteristics13=0.8e6, Wind_Characteristics14=0.9e6, Wind_Characteristics15=1, Wind_Characteristics16=1, Wind_Characteristics17=1, Wind_Characteristics18=1, Wind_Characteristics19=1, Wind_Characteristics20=1, Wind_Characteristics21=1, Wind_Characteristics22=1, Wind_Characteristics23=1, Wind_Characteristics24=1, Wind_Characteristics25=1, Wind_Characteristics26=[], Wind_Characteristics27=[], Wind_Characteristics28=[], Wind_Characteristics29=[], Wind_Characteristics30=[], Wind_Characteristics31=[], Wind_Characteristics32=[], Wind_Characteristics33=[], Wind_Characteristics34=[], Wind_Characteristics35=[], Power_Curve_Export=No, Visualization_save_PowerGraph_path='', Fault_Base_Duration_time_FRT=0.2, Fault_Ramp_End_Time_FRT=0.1, Fault_Base_Voltage_pu_FRT=0.1, Fault_End_Voltage_pu_FRT=0.85, FRT_Graph_Export=No, Visualization_save_FRT_path='', Ts=Ts}
      mask prompts: Nb_wt "Number of wind turbines [Nb_wt]"; Pnom "Wind turbine nominal power (W) [Pnom]"; Vgrid "Grid Voltage RMS (line-line) (V) [Vgrid]"; CutIn_Wind_Speed "Cut-in Wind Speed (m/s)"; Rated_Wind_Speed "Rated Wind Speed (m/s)"; CutOut_Wind_Speed "Cut-out Wind Speed (m/s)"; Power_Data_Filled "Was Power vs. Wind speed data obtained?"; Title "Wind Speed (m/s)"; Wind_Characteristics1 "1"; Wind_Characteristics2 "2"; Wind_Characteristics3 "3"; Wind_Characteristics4 "4"; Wind_Characteristics5 "5"; Wind_Characteristics6 "6"; Wind_Characteristics7 "7"; Wind_Characteristics8 "8"; Wind_Characteristics9 "9"; Wind_Characteristics10 "10"; Wind_Characteristics11 "11"; Wind_Characteristics12 "12"; Wind_Characteristics13 "13"; Wind_Characteristics14 "14"; Wind_Characteristics15 "15"; Wind_Characteristics16 "16"; Wind_Characteristics17 "17"; Wind_Characteristics18 "18"; Wind_Characteristics19 "19"; Wind_Characteristics20 "20"; Wind_Characteristics21 "21"; Wind_Characteristics22 "22"; Wind_Characteristics23 "23"; Wind_Characteristics24 "24"; Wind_Characteristics25 "25"; Wind_Characteristics26 "26"; Wind_Characteristics27 "27"; Wind_Characteristics28 "28"; Wind_Characteristics29 "29"; Wind_Characteristics30 "30"; Wind_Characteristics31 "31"; Wind_Characteristics32 "32"; Wind_Characteristics33 "33"; Wind_Characteristics34 "34"; Wind_Characteristics35 "35"; Power_Curve_Export "Export Power vs. Wind speed curve?"; Visualization_save_PowerGraph_path "Enter file path for the figures"; Fault_Base_Duration_time_FRT "Set base fault duration (Δs)"; Fault_Ramp_End_Time_FRT "Set post-fault ramp duration (Δs)"; Fault_Base_Voltage_pu_FRT "Set base voltage amplitude (p.u.)"; Fault_End_Voltage_pu_FRT "Set end voltage amplitude (p.u.)"; FRT_Graph_Export "Export FRT Code graph?"; Visualization_save_FRT_path "Enter file path for the figures"
      mask help: This block implements a model of a variable speed pitch controlled wind turbine using a synchronous generator.
      mask init: same as Versie2/SM_WT1/Wind Type IV Detailed v2.1 - 1
      mask TypeOptions CutIn_Wind_Speed: 1 | 2 | 3 | 4 | 5 | 6 | 7 | 8 | 9 | 10 | 11 | 12 | 13 | 14 | 15 | 16 | 17 | 18 | 19 | 20 | 21 | 22 | 23 | 24 | 25 | 26 | 27 | 28 | 29 | 30 | 31 | 32 | 33 | 34 | 35
      mask TypeOptions Rated_Wind_Speed: 1 | 2 | 3 | 4 | 5 | 6 | 7 | 8 | 9 | 10 | 11 | 12 | 13 | 14 | 15 | 16 | 17 | 18 | 19 | 20 | 21 | 22 | 23 | 24 | 25 | 26 | 27 | 28 | 29 | 30 | 31 | 32 | 33 | 34 | 35
      mask TypeOptions CutOut_Wind_Speed: 1 | 2 | 3 | 4 | 5 | 6 | 7 | 8 | 9 | 10 | 11 | 12 | 13 | 14 | 15 | 16 | 17 | 18 | 19 | 20 | 21 | 22 | 23 | 24 | 25 | 26 | 27 | 28 | 29 | 30 | 31 | 32 | 33 | 34 | 35
      mask TypeOptions Power_Data_Filled: Yes | No
      mask TypeOptions Power_Curve_Export: Print | Print and save | No
      mask TypeOptions FRT_Graph_Export: Print | Print and save | No
      mask DialogControl Container8 Prompt: General data
      mask DialogControl Container11 Prompt: Power data per turbine
      mask DialogControl Control2 Prompt: If no wind speed characteristics were found for the turbine the variables below may be set at their default values.
      mask DialogControl Power_Data_Table Prompt: If data for a certain wind speed is not found leave blank ([]). Power >= v_out and <=v_in shall not be filled.
      mask DialogControl Container16 Prompt: Fault ride through settings
      mask DialogControl Container17 Prompt: Time variables
      mask DialogControl Container18 Prompt: Voltage thresholds
      mask Display: image('windturbine4.jpg')
  Wind Type IV Detailed v2.1 - 24 : Subsystem  LoadFcn=%find_system(gcs,'FollowLinks', 'on', 'LookUnderMasks', 'all');  mask(Wind Turbine: Model 7){Nb_wt=26, Pnom=15e6, Vgrid=66000, CutIn_Wind_Speed=3, Rated_Wind_Speed=12, CutOut_Wind_Speed=25, Power_Data_Filled=No, Title=Power Data (W), Wind_Characteristics1=0, Wind_Characteristics2=0, Wind_Characteristics3=0, Wind_Characteristics4=0, Wind_Characteristics5=0, Wind_Characteristics6=0.1e6, Wind_Characteristics7=0.2e6, Wind_Characteristics8=0.3e6, Wind_Characteristics9=0.4e6, Wind_Characteristics10=0.5e6, Wind_Characteristics11=0.6e6, Wind_Characteristics12=0.7e6, Wind_Characteristics13=0.8e6, Wind_Characteristics14=0.9e6, Wind_Characteristics15=1, Wind_Characteristics16=1, Wind_Characteristics17=1, Wind_Characteristics18=1, Wind_Characteristics19=1, Wind_Characteristics20=1, Wind_Characteristics21=1, Wind_Characteristics22=1, Wind_Characteristics23=1, Wind_Characteristics24=1, Wind_Characteristics25=1, Wind_Characteristics26=[], Wind_Characteristics27=[], Wind_Characteristics28=[], Wind_Characteristics29=[], Wind_Characteristics30=[], Wind_Characteristics31=[], Wind_Characteristics32=[], Wind_Characteristics33=[], Wind_Characteristics34=[], Wind_Characteristics35=[], Power_Curve_Export=No, Visualization_save_PowerGraph_path='', Fault_Base_Duration_time_FRT=0.2, Fault_Ramp_End_Time_FRT=0.1, Fault_Base_Voltage_pu_FRT=0.1, Fault_End_Voltage_pu_FRT=0.85, FRT_Graph_Export=No, Visualization_save_FRT_path='', Ts=Ts}
      mask prompts: Nb_wt "Number of wind turbines [Nb_wt]"; Pnom "Wind turbine nominal power (W) [Pnom]"; Vgrid "Grid Voltage RMS (line-line) (V) [Vgrid]"; CutIn_Wind_Speed "Cut-in Wind Speed (m/s)"; Rated_Wind_Speed "Rated Wind Speed (m/s)"; CutOut_Wind_Speed "Cut-out Wind Speed (m/s)"; Power_Data_Filled "Was Power vs. Wind speed data obtained?"; Title "Wind Speed (m/s)"; Wind_Characteristics1 "1"; Wind_Characteristics2 "2"; Wind_Characteristics3 "3"; Wind_Characteristics4 "4"; Wind_Characteristics5 "5"; Wind_Characteristics6 "6"; Wind_Characteristics7 "7"; Wind_Characteristics8 "8"; Wind_Characteristics9 "9"; Wind_Characteristics10 "10"; Wind_Characteristics11 "11"; Wind_Characteristics12 "12"; Wind_Characteristics13 "13"; Wind_Characteristics14 "14"; Wind_Characteristics15 "15"; Wind_Characteristics16 "16"; Wind_Characteristics17 "17"; Wind_Characteristics18 "18"; Wind_Characteristics19 "19"; Wind_Characteristics20 "20"; Wind_Characteristics21 "21"; Wind_Characteristics22 "22"; Wind_Characteristics23 "23"; Wind_Characteristics24 "24"; Wind_Characteristics25 "25"; Wind_Characteristics26 "26"; Wind_Characteristics27 "27"; Wind_Characteristics28 "28"; Wind_Characteristics29 "29"; Wind_Characteristics30 "30"; Wind_Characteristics31 "31"; Wind_Characteristics32 "32"; Wind_Characteristics33 "33"; Wind_Characteristics34 "34"; Wind_Characteristics35 "35"; Power_Curve_Export "Export Power vs. Wind speed curve?"; Visualization_save_PowerGraph_path "Enter file path for the figures"; Fault_Base_Duration_time_FRT "Set base fault duration (Δs)"; Fault_Ramp_End_Time_FRT "Set post-fault ramp duration (Δs)"; Fault_Base_Voltage_pu_FRT "Set base voltage amplitude (p.u.)"; Fault_End_Voltage_pu_FRT "Set end voltage amplitude (p.u.)"; FRT_Graph_Export "Export FRT Code graph?"; Visualization_save_FRT_path "Enter file path for the figures"
      mask help: This block implements a model of a variable speed pitch controlled wind turbine using a synchronous generator.
      mask init: same as Versie2/SM_WT1/Wind Type IV Detailed v2.1 - 1
      mask TypeOptions CutIn_Wind_Speed: 1 | 2 | 3 | 4 | 5 | 6 | 7 | 8 | 9 | 10 | 11 | 12 | 13 | 14 | 15 | 16 | 17 | 18 | 19 | 20 | 21 | 22 | 23 | 24 | 25 | 26 | 27 | 28 | 29 | 30 | 31 | 32 | 33 | 34 | 35
      mask TypeOptions Rated_Wind_Speed: 1 | 2 | 3 | 4 | 5 | 6 | 7 | 8 | 9 | 10 | 11 | 12 | 13 | 14 | 15 | 16 | 17 | 18 | 19 | 20 | 21 | 22 | 23 | 24 | 25 | 26 | 27 | 28 | 29 | 30 | 31 | 32 | 33 | 34 | 35
      mask TypeOptions CutOut_Wind_Speed: 1 | 2 | 3 | 4 | 5 | 6 | 7 | 8 | 9 | 10 | 11 | 12 | 13 | 14 | 15 | 16 | 17 | 18 | 19 | 20 | 21 | 22 | 23 | 24 | 25 | 26 | 27 | 28 | 29 | 30 | 31 | 32 | 33 | 34 | 35
      mask TypeOptions Power_Data_Filled: Yes | No
      mask TypeOptions Power_Curve_Export: Print | Print and save | No
      mask TypeOptions FRT_Graph_Export: Print | Print and save | No
      mask DialogControl Container8 Prompt: General data
      mask DialogControl Container11 Prompt: Power data per turbine
      mask DialogControl Control2 Prompt: If no wind speed characteristics were found for the turbine the variables below may be set at their default values.
      mask DialogControl Power_Data_Table Prompt: If data for a certain wind speed is not found leave blank ([]). Power >= v_out and <=v_in shall not be filled.
      mask DialogControl Container16 Prompt: Fault ride through settings
      mask DialogControl Container17 Prompt: Time variables
      mask DialogControl Container18 Prompt: Voltage thresholds
      mask Display: image('windturbine4.jpg')
  Wind Type IV Detailed v2.1 - 3 : Subsystem  Commented=on  LoadFcn=%find_system(gcs,'FollowLinks', 'on', 'LookUnderMasks', 'all');  mask(Wind Turbine: Model 7){Nb_wt=10, Pnom=15e6, Vgrid=66000, CutIn_Wind_Speed=3, Rated_Wind_Speed=12, CutOut_Wind_Speed=25, Power_Data_Filled=No, Title=Power Data (W), Wind_Characteristics1=0, Wind_Characteristics2=0, Wind_Characteristics3=0, Wind_Characteristics4=0, Wind_Characteristics5=0, Wind_Characteristics6=0.1e6, Wind_Characteristics7=0.2e6, Wind_Characteristics8=0.3e6, Wind_Characteristics9=0.4e6, Wind_Characteristics10=0.5e6, Wind_Characteristics11=0.6e6, Wind_Characteristics12=0.7e6, Wind_Characteristics13=0.8e6, Wind_Characteristics14=0.9e6, Wind_Characteristics15=1, Wind_Characteristics16=1, Wind_Characteristics17=1, Wind_Characteristics18=1, Wind_Characteristics19=1, Wind_Characteristics20=1, Wind_Characteristics21=1, Wind_Characteristics22=1, Wind_Characteristics23=1, Wind_Characteristics24=1, Wind_Characteristics25=1, Wind_Characteristics26=[], Wind_Characteristics27=[], Wind_Characteristics28=[], Wind_Characteristics29=[], Wind_Characteristics30=[], Wind_Characteristics31=[], Wind_Characteristics32=[], Wind_Characteristics33=[], Wind_Characteristics34=[], Wind_Characteristics35=[], Power_Curve_Export=No, Visualization_save_PowerGraph_path='', Fault_Base_Duration_time_FRT=0.2, Fault_Ramp_End_Time_FRT=0.1, Fault_Base_Voltage_pu_FRT=0.1, Fault_End_Voltage_pu_FRT=0.85, FRT_Graph_Export=No, Visualization_save_FRT_path='', Ts=Ts}
      mask prompts: Nb_wt "Number of wind turbines [Nb_wt]"; Pnom "Wind turbine nominal power (W) [Pnom]"; Vgrid "Grid Voltage RMS (line-line) (V) [Vgrid]"; CutIn_Wind_Speed "Cut-in Wind Speed (m/s)"; Rated_Wind_Speed "Rated Wind Speed (m/s)"; CutOut_Wind_Speed "Cut-out Wind Speed (m/s)"; Power_Data_Filled "Was Power vs. Wind speed data obtained?"; Title "Wind Speed (m/s)"; Wind_Characteristics1 "1"; Wind_Characteristics2 "2"; Wind_Characteristics3 "3"; Wind_Characteristics4 "4"; Wind_Characteristics5 "5"; Wind_Characteristics6 "6"; Wind_Characteristics7 "7"; Wind_Characteristics8 "8"; Wind_Characteristics9 "9"; Wind_Characteristics10 "10"; Wind_Characteristics11 "11"; Wind_Characteristics12 "12"; Wind_Characteristics13 "13"; Wind_Characteristics14 "14"; Wind_Characteristics15 "15"; Wind_Characteristics16 "16"; Wind_Characteristics17 "17"; Wind_Characteristics18 "18"; Wind_Characteristics19 "19"; Wind_Characteristics20 "20"; Wind_Characteristics21 "21"; Wind_Characteristics22 "22"; Wind_Characteristics23 "23"; Wind_Characteristics24 "24"; Wind_Characteristics25 "25"; Wind_Characteristics26 "26"; Wind_Characteristics27 "27"; Wind_Characteristics28 "28"; Wind_Characteristics29 "29"; Wind_Characteristics30 "30"; Wind_Characteristics31 "31"; Wind_Characteristics32 "32"; Wind_Characteristics33 "33"; Wind_Characteristics34 "34"; Wind_Characteristics35 "35"; Power_Curve_Export "Export Power vs. Wind speed curve?"; Visualization_save_PowerGraph_path "Enter file path for the figures"; Fault_Base_Duration_time_FRT "Set base fault duration (Δs)"; Fault_Ramp_End_Time_FRT "Set post-fault ramp duration (Δs)"; Fault_Base_Voltage_pu_FRT "Set base voltage amplitude (p.u.)"; Fault_End_Voltage_pu_FRT "Set end voltage amplitude (p.u.)"; FRT_Graph_Export "Export FRT Code graph?"; Visualization_save_FRT_path "Enter file path for the figures"
      mask help: This block implements a model of a variable speed pitch controlled wind turbine using a synchronous generator.
      mask init: same as Versie2/SM_WT1/Wind Type IV Detailed v2.1 - 1
      mask TypeOptions CutIn_Wind_Speed: 1 | 2 | 3 | 4 | 5 | 6 | 7 | 8 | 9 | 10 | 11 | 12 | 13 | 14 | 15 | 16 | 17 | 18 | 19 | 20 | 21 | 22 | 23 | 24 | 25 | 26 | 27 | 28 | 29 | 30 | 31 | 32 | 33 | 34 | 35
      mask TypeOptions Rated_Wind_Speed: 1 | 2 | 3 | 4 | 5 | 6 | 7 | 8 | 9 | 10 | 11 | 12 | 13 | 14 | 15 | 16 | 17 | 18 | 19 | 20 | 21 | 22 | 23 | 24 | 25 | 26 | 27 | 28 | 29 | 30 | 31 | 32 | 33 | 34 | 35
      mask TypeOptions CutOut_Wind_Speed: 1 | 2 | 3 | 4 | 5 | 6 | 7 | 8 | 9 | 10 | 11 | 12 | 13 | 14 | 15 | 16 | 17 | 18 | 19 | 20 | 21 | 22 | 23 | 24 | 25 | 26 | 27 | 28 | 29 | 30 | 31 | 32 | 33 | 34 | 35
      mask TypeOptions Power_Data_Filled: Yes | No
      mask TypeOptions Power_Curve_Export: Print | Print and save | No
      mask TypeOptions FRT_Graph_Export: Print | Print and save | No
      mask DialogControl Container8 Prompt: General data
      mask DialogControl Container11 Prompt: Power data per turbine
      mask DialogControl Control2 Prompt: If no wind speed characteristics were found for the turbine the variables below may be set at their default values.
      mask DialogControl Power_Data_Table Prompt: If data for a certain wind speed is not found leave blank ([]). Power >= v_out and <=v_in shall not be filled.
      mask DialogControl Container16 Prompt: Fault ride through settings
      mask DialogControl Container17 Prompt: Time variables
      mask DialogControl Container18 Prompt: Voltage thresholds
      mask Display: image('windturbine4.jpg')
  Wind Type IV Detailed v2.1 - 33 : Subsystem  LoadFcn=%find_system(gcs,'FollowLinks', 'on', 'LookUnderMasks', 'all');  mask(Wind Turbine: Model 7){Nb_wt=24, Pnom=15e6, Vgrid=66000, CutIn_Wind_Speed=3, Rated_Wind_Speed=12, CutOut_Wind_Speed=25, Power_Data_Filled=No, Title=Power Data (W), Wind_Characteristics1=0, Wind_Characteristics2=0, Wind_Characteristics3=0, Wind_Characteristics4=0, Wind_Characteristics5=0, Wind_Characteristics6=0.1e6, Wind_Characteristics7=0.2e6, Wind_Characteristics8=0.3e6, Wind_Characteristics9=0.4e6, Wind_Characteristics10=0.5e6, Wind_Characteristics11=0.6e6, Wind_Characteristics12=0.7e6, Wind_Characteristics13=0.8e6, Wind_Characteristics14=0.9e6, Wind_Characteristics15=1, Wind_Characteristics16=1, Wind_Characteristics17=1, Wind_Characteristics18=1, Wind_Characteristics19=1, Wind_Characteristics20=1, Wind_Characteristics21=1, Wind_Characteristics22=1, Wind_Characteristics23=1, Wind_Characteristics24=1, Wind_Characteristics25=1, Wind_Characteristics26=[], Wind_Characteristics27=[], Wind_Characteristics28=[], Wind_Characteristics29=[], Wind_Characteristics30=[], Wind_Characteristics31=[], Wind_Characteristics32=[], Wind_Characteristics33=[], Wind_Characteristics34=[], Wind_Characteristics35=[], Power_Curve_Export=No, Visualization_save_PowerGraph_path='', Fault_Base_Duration_time_FRT=0.2, Fault_Ramp_End_Time_FRT=0.1, Fault_Base_Voltage_pu_FRT=0.1, Fault_End_Voltage_pu_FRT=0.85, FRT_Graph_Export=No, Visualization_save_FRT_path='', Ts=Ts}
      mask prompts: Nb_wt "Number of wind turbines [Nb_wt]"; Pnom "Wind turbine nominal power (W) [Pnom]"; Vgrid "Grid Voltage RMS (line-line) (V) [Vgrid]"; CutIn_Wind_Speed "Cut-in Wind Speed (m/s)"; Rated_Wind_Speed "Rated Wind Speed (m/s)"; CutOut_Wind_Speed "Cut-out Wind Speed (m/s)"; Power_Data_Filled "Was Power vs. Wind speed data obtained?"; Title "Wind Speed (m/s)"; Wind_Characteristics1 "1"; Wind_Characteristics2 "2"; Wind_Characteristics3 "3"; Wind_Characteristics4 "4"; Wind_Characteristics5 "5"; Wind_Characteristics6 "6"; Wind_Characteristics7 "7"; Wind_Characteristics8 "8"; Wind_Characteristics9 "9"; Wind_Characteristics10 "10"; Wind_Characteristics11 "11"; Wind_Characteristics12 "12"; Wind_Characteristics13 "13"; Wind_Characteristics14 "14"; Wind_Characteristics15 "15"; Wind_Characteristics16 "16"; Wind_Characteristics17 "17"; Wind_Characteristics18 "18"; Wind_Characteristics19 "19"; Wind_Characteristics20 "20"; Wind_Characteristics21 "21"; Wind_Characteristics22 "22"; Wind_Characteristics23 "23"; Wind_Characteristics24 "24"; Wind_Characteristics25 "25"; Wind_Characteristics26 "26"; Wind_Characteristics27 "27"; Wind_Characteristics28 "28"; Wind_Characteristics29 "29"; Wind_Characteristics30 "30"; Wind_Characteristics31 "31"; Wind_Characteristics32 "32"; Wind_Characteristics33 "33"; Wind_Characteristics34 "34"; Wind_Characteristics35 "35"; Power_Curve_Export "Export Power vs. Wind speed curve?"; Visualization_save_PowerGraph_path "Enter file path for the figures"; Fault_Base_Duration_time_FRT "Set base fault duration (Δs)"; Fault_Ramp_End_Time_FRT "Set post-fault ramp duration (Δs)"; Fault_Base_Voltage_pu_FRT "Set base voltage amplitude (p.u.)"; Fault_End_Voltage_pu_FRT "Set end voltage amplitude (p.u.)"; FRT_Graph_Export "Export FRT Code graph?"; Visualization_save_FRT_path "Enter file path for the figures"
      mask help: This block implements a model of a variable speed pitch controlled wind turbine using a synchronous generator.
      mask init: same as Versie2/SM_WT1/Wind Type IV Detailed v2.1 - 1
      mask TypeOptions CutIn_Wind_Speed: 1 | 2 | 3 | 4 | 5 | 6 | 7 | 8 | 9 | 10 | 11 | 12 | 13 | 14 | 15 | 16 | 17 | 18 | 19 | 20 | 21 | 22 | 23 | 24 | 25 | 26 | 27 | 28 | 29 | 30 | 31 | 32 | 33 | 34 | 35
      mask TypeOptions Rated_Wind_Speed: 1 | 2 | 3 | 4 | 5 | 6 | 7 | 8 | 9 | 10 | 11 | 12 | 13 | 14 | 15 | 16 | 17 | 18 | 19 | 20 | 21 | 22 | 23 | 24 | 25 | 26 | 27 | 28 | 29 | 30 | 31 | 32 | 33 | 34 | 35
      mask TypeOptions CutOut_Wind_Speed: 1 | 2 | 3 | 4 | 5 | 6 | 7 | 8 | 9 | 10 | 11 | 12 | 13 | 14 | 15 | 16 | 17 | 18 | 19 | 20 | 21 | 22 | 23 | 24 | 25 | 26 | 27 | 28 | 29 | 30 | 31 | 32 | 33 | 34 | 35
      mask TypeOptions Power_Data_Filled: Yes | No
      mask TypeOptions Power_Curve_Export: Print | Print and save | No
      mask TypeOptions FRT_Graph_Export: Print | Print and save | No
      mask DialogControl Container8 Prompt: General data
      mask DialogControl Container11 Prompt: Power data per turbine
      mask DialogControl Control2 Prompt: If no wind speed characteristics were found for the turbine the variables below may be set at their default values.
      mask DialogControl Power_Data_Table Prompt: If data for a certain wind speed is not found leave blank ([]). Power >= v_out and <=v_in shall not be filled.
      mask DialogControl Container16 Prompt: Fault ride through settings
      mask DialogControl Container17 Prompt: Time variables
      mask DialogControl Container18 Prompt: Voltage thresholds
      mask Display: image('windturbine4.jpg')
  Turbine_Measurements : Outport  VectorParamsAs1DForOutWhenUnconnected=on
  Bus_Measurements : Outport  Port=2  VectorParamsAs1DForOutWhenUnconnected=on
  Trip : Outport  Port=3  VectorParamsAs1DForOutWhenUnconnected=on
  Fault : Outport  Port=4  VectorParamsAs1DForOutWhenUnconnected=on
  wires:
  Fault_timing_generator/2(acqu) -> Terminator1/1
  [fault_params] -> Fault_timing_generator/1(fault_params)
  Unit Delay/1 -> [fault_trigger]
  Fault_timing_generator/1(fault) -> Unit Delay/1
  Constant3/1 -> Fault_timing_generator/2(pulse)
  Qref_pu1/1 -> Wind Type IV Detailed v2.1 - 1/2(Qref_pu)
  [wind] -> Wind Type IV Detailed v2.1 - 1/1("Wind (m/s) ")
  [Trip] -> Trip/1  "Trip"
  [WindFarm_Selection_1] -> Multiport Switch/2  "WindFarm_Selection_1"
  [WindFarm_Selection_2] -> Multiport Switch/3  "WindFarm_Selection_2"
  [WindFarm_Selection_3] -> Multiport Switch/4  "WindFarm_Selection_3"
  [WindFarm_Selection_4] -> Multiport Switch/5  "WindFarm_Selection_4"
  [WindFarm_Selection_5] -> Multiport Switch/6  "WindFarm_Selection_5"
  [WindFarm_Selection_6] -> Multiport Switch/7  "WindFarm_Selection_6"
  [WindFarm_Selection_7] -> Multiport Switch/8  "WindFarm_Selection_7"
  [WindFarm_Selection_8] -> Multiport Switch/9  "WindFarm_Selection_8"
  [WindFarm_Selection_9] -> Multiport Switch/10  "WindFarm_Selection_9"
  [WindFarm_Selection_10] -> Multiport Switch/11  "WindFarm_Selection_10"
  [BusD] -> Multiport Switch1/5  "BusD"
  [BusC] -> Multiport Switch1/4  "BusC"
  [BusB] -> Multiport Switch1/3  "BusB"
  [BusA] -> Multiport Switch1/2  "BusA"
  BusC/1(Vabc) -> Subsystem2/1(V)  "Vabc"
  BusC/2(Iabc) -> Subsystem2/2(I)  "Iabc"
  Subsystem2/1(Out1) -> Bus Selector1/1
  "Dummy Bus Signals "/1(Out1) -> [BusC], [BusB], [BusD]
  Multiport Switch/1 -> Turbine_Measurements/1
  Multiport Switch1/1 -> Bus_Measurements/1
  wind/1 -> [wind]
  [TurbineSelection] -> Multiport Switch/1
  Bus_Fault/1 -> [Fault_Iabc]
  [Fault_Iabc] -> Fault/1  "Trip"
  [BusSelection] -> Multiport Switch1/1
  [fault_trigger] -> Three-Phase Fault/1
  "FaultParams "/1 -> [fault_params]
  [wind] -> Wind Type IV Detailed v2.1 - 2/1("Wind (m/s) ")
  Qref_pu3/1 -> Wind Type IV Detailed v2.1 - 2/2(Qref_pu)
  Dummy WF signals/1(m) -> [WindFarm_Selection_8], [WindFarm_Selection_7], [WindFarm_Selection_6], [WindFarm_Selection_5], [WindFarm_Selection_1], [WindFarm_Selection_2], [WindFarm_Selection_3], [WindFarm_Selection_4], [WindFarm_Selection_9], [WindFarm_Selection_10]
  Subsystem1/1(Out1) -> [BusA]
  Qref_pu2/1 -> Wind Type IV Detailed v2.1 - 3/2(Qref_pu)
  From3/1 -> Wind Type IV Detailed v2.1 - 3/1("Wind (m/s) ")
  Wind Type IV Detailed v2.1 - 3/1(m) -> ?
  BusB/1(Vabc) -> Subsystem3/1(V)  "Vabc"
  BusB/2(Iabc) -> Subsystem3/2(I)  "Iabc"
  BusD/2(Iabc) -> Subsystem4/2(I)  "Iabc"
  BusD/1(Vabc) -> Subsystem4/1(V)  "Vabc"
  PlotSelection/1 -> Bus Selector/1
  Bus Selector/2 -> [BusSelection]  "<Bus>"
  Bus Selector/1 -> [TurbineSelection]  "<Turbine>"
  Bus Selector1/2 -> Scope1/2  "<Iabc>"
  Bus Selector1/1 -> Scope1/1  "<Vabc>"
  Bus Selector1/3 -> Scope1/3  "<PQ>"
  Bus Selector2/3 -> Scope2/3  "<PQ>"
  Bus Selector2/1 -> Scope2/1  "<Vabc>"
  Bus Selector2/2 -> Scope2/2  "<Iabc>"
  [BusA] -> Bus Selector2/1
  From19/1 -> Differential Element 1/2(Iabc Local)
  From11/1 -> Differential Element 2/3(Vabc Local)
  Overcurrent Element 1/1(Trip) -> Goto6/1
  From37/1 -> Bus Creator/3  "Z"
  Bus Creator1/1 -> Goto39/1, Scope Bus2/3  "Trip"
  Step/1 -> Goto33/1
  From18/1 -> Differential Element 2/1(Iabc Remote)
  Differential Element 2/1(Trip) -> Goto23/1
  From9/1 -> Overcurrent Element 1/1(Iabc)
  From36/1 -> Bus Creator/2  "Diff"
  Impedance Element 2/1(Trip) -> Goto24/1
  Impedance Element 1/1(Trip) -> Goto27/1
  From8/1 -> Transformer differential element 1/2(IX)
  From42/1 -> Impedance Element 2/2(Iabc)
  From40/1 -> Impedance Element 2/1(Vabc)
  From59/1 -> Differential Element 1/3(Vabc Local)
  From33/1 -> Scope Bus2/1  "I"
  Bus Creator/1 -> Goto35/1, Scope Bus1/3  "Trip"
  From35/1 -> Bus Creator/1  "OC"
  From50/1 -> Overcurrent Element 2/Enable
  From30/1 -> Differential Element 1/1(Iabc Remote)
  From53/1 -> Transformer differential element 1/Enable
  From47/1 -> Scope Bus1/1  "I"
  From17/1 -> Differential Element 2/2(Iabc Local)
  From49/1 -> Impedance Element 1/Enable
  From52/1 -> Impedance Element 2/Enable
  Overcurrent Element 2/1(Trip) -> Goto7/1
  Differential Element 1/1(Trip) -> Goto26/1
  From38/1 -> Impedance Element 1/2(Iabc)
  From48/1 -> Scope Bus1/2  "V"
  From34/1 -> Scope Bus2/2  "V"
  From55/1 -> Scope Bus4/1, Scope Bus3/1
  From39/1 -> Impedance Element 1/1(Vabc)
  From45/1 -> Bus Creator1/2  "Diff"
  Transformer differential element 1/1(Trip) -> Goto25/1
  From57/1 -> Scope Bus4/3
  From32/1 -> Transformer differential element 1/1(IH)
  From44/1 -> Bus Creator1/1  "OC"
  From54/1 -> Scope Bus3/2
  From56/1 -> Scope Bus4/2
  From46/1 -> Bus Creator1/3  "Z"
  From58/1 -> Overcurrent Element 1/Enable
  From51/1 -> Differential Element 2/Enable
  From10/1 -> Differential Element 1/Enable
  From43/1 -> Goto37/1, Scope Bus3/3  "Diff"
  From31/1 -> Overcurrent Element 2/1(Iabc)
  CT-ratio/1 -> [I_1]
  BusC1/2(Iabc) -> CT-ratio/1  "Iabc"
  VT-ratio/1 -> [V_1]
  BusC1/1(Vabc) -> VT-ratio/1  "Vabc"
  VT-ratio1/1 -> [V_2]
  CT-ratio1/1 -> [I_2]
  BusA/2(Iabc) -> CT-ratio1/1, Subsystem1/2(I)  "Iabc"
  BusA/1(Vabc) -> VT-ratio1/1, Subsystem1/1(V)  "Vabc"
  BusC2/1(Vabc) -> VT-ratio2/1  "Vabc"
  VT-ratio2/1 -> [V_3]
  CT-ratio2/1 -> [I_3]
  BusC2/2(Iabc) -> CT-ratio2/1  "Iabc"
  OR/1 -> Goto36/1
  From60/1 -> OR/1
  From61/1 -> OR/2
  From62/1 -> OR/3
  From63/1 -> Overcurrent Inverse time/1(Iabc)
  Overcurrent Inverse time/1(Trip) -> Goto40/1
  From66/1 -> Overcurrent Inverse time/Enable
  From64/1 -> Bus Creator/4  "Z"
  Bus Selector3/1 -> Scope3/1  "<Vabc>"
  Subsystem5/1(Out1) -> Bus Selector3/1
  BusC3/1(Vabc) -> Subsystem5/1(V)  "Vabc"
  Bus Selector3/3 -> Scope3/3  "<PQ>"
  Bus Selector3/2 -> Scope3/2  "<Iabc>"
  BusC3/2(Iabc) -> Subsystem5/2(I)  "Iabc"
  [wind] -> Wind Type IV Detailed v2.1 - 11/1("Wind (m/s) ")
  Qref_pu11/1 -> Wind Type IV Detailed v2.1 - 11/2(Qref_pu)
  [wind] -> Wind Type IV Detailed v2.1 - 14/1("Wind (m/s) ")
  BusC4/2(Iabc) -> Subsystem6/2(I)  "Iabc"
  Bus Selector4/3 -> Scope4/3  "<PQ>"
  Subsystem6/1(Out1) -> Bus Selector4/1
  BusC4/1(Vabc) -> Subsystem6/1(V)  "Vabc"
  Bus Selector4/2 -> Scope4/2  "<Iabc>"
  Bus Selector4/1 -> Scope4/1  "<Vabc>"
  Qref_pu14/1 -> Wind Type IV Detailed v2.1 - 14/2(Qref_pu)
  Qref_pu24/1 -> Wind Type IV Detailed v2.1 - 24/2(Qref_pu)
  Bus Selector6/1 -> Scope6/1  "<Vabc>"
  Subsystem8/1(Out1) -> Bus Selector6/1
  Bus Selector6/2 -> Scope6/2  "<Iabc>"
  BusC6/1(Vabc) -> Subsystem8/1(V)  "Vabc"
  [wind] -> Wind Type IV Detailed v2.1 - 24/1("Wind (m/s) ")
  BusC5/2(Iabc) -> Subsystem7/2(I)  "Iabc"
  Bus Selector5/3 -> Scope5/3  "<PQ>"
  Subsystem7/1(Out1) -> Bus Selector5/1
  BusC5/1(Vabc) -> Subsystem7/1(V)  "Vabc"
  Bus Selector5/2 -> Scope5/2  "<Iabc>"
  Bus Selector5/1 -> Scope5/1  "<Vabc>"
  Bus Selector6/3 -> Scope6/3  "<PQ>"
  BusC6/2(Iabc) -> Subsystem8/2(I)  "Iabc"
  Qref_pu33/1 -> Wind Type IV Detailed v2.1 - 33/2(Qref_pu)
  [wind] -> Wind Type IV Detailed v2.1 - 33/1("Wind (m/s) ")
  BusC7/1(Vabc) -> Subsystem9/1(V)  "Vabc"
  BusC7/2(Iabc) -> Subsystem9/2(I)  "Iabc"
  Bus Selector7/3 -> Scope7/3  "<PQ>"
  Bus Selector7/2 -> Scope7/2  "<Iabc>"
  Bus Selector7/1 -> Scope7/1  "<Vabc>"
  Subsystem9/1(Out1) -> Bus Selector7/1
  Bus Selector8/1 -> Scope8/1  "<Vabc>"
  Bus Selector8/2 -> Scope8/2  "<Iabc>"
  Bus Selector8/3 -> Scope8/3  "<PQ>"
  BusC8/2(Iabc) -> Subsystem10/2(I)  "Iabc"
  BusC8/1(Vabc) -> Subsystem10/1(V)  "Vabc"
  Subsystem10/1(Out1) -> Bus Selector8/1
  Bus Selector9/1 -> Scope9/1  "<Vabc>"
  Bus Selector9/2 -> Scope9/2  "<Iabc>"
  Bus Selector9/3 -> Scope9/3  "<PQ>"
  BusC9/2(Iabc) -> Subsystem11/2(I)  "Iabc"
  BusC9/1(Vabc) -> Subsystem11/1(V)  "Vabc"
  Subsystem11/1(Out1) -> Bus Selector9/1
  Bus Selector10/1 -> Scope10/1  "<Vabc>"
  Bus Selector10/2 -> Scope10/2  "<Iabc>"
  Bus Selector10/3 -> Scope10/3  "<PQ>"
  BusC10/2(Iabc) -> Subsystem12/2(I)  "Iabc"
  BusC10/1(Vabc) -> Subsystem12/1(V)  "Vabc"
  Subsystem12/1(Out1) -> Bus Selector10/1
  Bus Selector11/1 -> Scope11/1  "<Vabc>"
  Bus Selector11/2 -> Scope11/2  "<Iabc>"
  Bus Selector11/3 -> Scope11/3  "<PQ>"
  BusC11/2(Iabc) -> Subsystem13/2(I)  "Iabc"
  BusC11/1(Vabc) -> Subsystem13/1(V)  "Vabc"
  Subsystem13/1(Out1) -> Bus Selector11/1
  Subsystem14/1(Out1) -> Bus Selector12/1
  BusC12/1(Vabc) -> Subsystem14/1(V)  "Vabc"
  Bus Selector12/2 -> Scope12/2  "<Iabc>"
  BusC12/2(Iabc) -> Subsystem14/2(I)  "Iabc"
  Bus Selector12/1 -> Scope12/1  "<Vabc>"
  Bus Selector12/3 -> Scope12/3  "<PQ>"
  BusC13/2(Iabc) -> Subsystem15/2(I)  "Iabc"
  Bus Selector13/1 -> Scope13/1  "<Vabc>"
  Bus Selector13/3 -> Scope13/3  "<PQ>"
  Bus Selector13/2 -> Scope13/2  "<Iabc>"
  BusC13/1(Vabc) -> Subsystem15/1(V)  "Vabc"
  Subsystem15/1(Out1) -> Bus Selector13/1
  BusC14/2(Iabc) -> Subsystem16/2(I)  "Iabc"
  Bus Selector14/1 -> Scope14/1  "<Vabc>"
  Bus Selector14/3 -> Scope14/3  "<PQ>"
  Bus Selector14/2 -> Scope14/2  "<Iabc>"
  BusC14/1(Vabc) -> Subsystem16/1(V)  "Vabc"
  Subsystem16/1(Out1) -> Bus Selector14/1
  BusC15/2(Iabc) -> Subsystem17/2(I)  "Iabc"
  Bus Selector15/1 -> Scope15/1  "<Vabc>"
  Bus Selector15/3 -> Scope15/3  "<PQ>"
  Bus Selector15/2 -> Scope15/2  "<Iabc>"
  BusC15/1(Vabc) -> Subsystem17/1(V)  "Vabc"
  Subsystem17/1(Out1) -> Bus Selector15/1
  BusC16/2(Iabc) -> Subsystem18/2(I)  "Iabc"
  Bus Selector16/1 -> Scope16/1  "<Vabc>"
  Bus Selector16/3 -> Scope16/3  "<PQ>"
  Bus Selector16/2 -> Scope16/2  "<Iabc>"
  BusC16/1(Vabc) -> Subsystem18/1(V)  "Vabc"
  Subsystem18/1(Out1) -> Bus Selector16/1
  BusC17/2(Iabc) -> Subsystem19/2(I)  "Iabc"
  Bus Selector17/1 -> Scope17/1  "<Vabc>"
  Bus Selector17/3 -> Scope17/3  "<PQ>"
  Bus Selector17/2 -> Scope17/2  "<Iabc>"
  BusC17/1(Vabc) -> Subsystem19/1(V)  "Vabc"
  Subsystem19/1(Out1) -> Bus Selector17/1
  connections:
  5 km series1/LConn1 -- BusC1/LConn1 -- 2500 MVA X0/X1=1/RConn1
  5 km series1/LConn2 -- BusC1/LConn2 -- 2500 MVA X0/X1=1/RConn2
  Ground2/LConn1 -- Vac kV1/LConn1
  2500 MVA X0/X1=1/LConn2 -- Vac kV1/RConn2
  2500 MVA X0/X1=1/LConn3 -- Vac kV1/RConn3
  Vac kV1/RConn1 -- 2500 MVA X0/X1=1/LConn1
  5 km series2/LConn1 -- 5 km series1/RConn1
  5 km series1/RConn2 -- 5 km series2/LConn2
  5 km series2/LConn3 -- 5 km series1/RConn3
  2500 MVA X0/X1=1/RConn3 -- BusC1/LConn3 -- 5 km series1/LConn3
  " 1"/LConn1 -- 5 km series2/RConn1
  " 1"/LConn2 -- 5 km series2/RConn2
  5 km series2/RConn3 -- " 1"/LConn3
  BusC/LConn1 -- " 1"/RConn1
  BusC/LConn3 -- " 1"/RConn3
  BusC/LConn2 -- " 1"/RConn2
  5 km fault2/LConn2 -- 5 km fault1/RConn2 -- Bus_Fault/LConn2
  Bus_Fault/RConn2 -- Three-Phase Fault/LConn2 -- Controllable Fault/RConn2
  5 km fault2/LConn3 -- 5 km fault1/RConn3 -- Bus_Fault/LConn3
  Bus_Fault/RConn3 -- Controllable Fault/RConn3 -- Three-Phase Fault/LConn3
  5 km fault2/LConn1 -- 5 km fault1/RConn1 -- Bus_Fault/LConn1
  Bus_Fault/RConn1 -- Controllable Fault/RConn1 -- Three-Phase Fault/LConn1
  "Three-Phase Breaker "/RConn2 -- 5 km fault1/LConn2
  5 km fault2/RConn1 -- Three-Phase Breaker 4/LConn1
  "Three-Phase Breaker "/RConn1 -- 5 km fault1/LConn1
  5 km fault2/RConn2 -- Three-Phase Breaker 4/LConn2
  5 km fault2/RConn3 -- Three-Phase Breaker 4/LConn3
  "Three-Phase Breaker "/RConn3 -- 5 km fault1/LConn3
  " 2"/LConn3 -- BusA/RConn3
  " 2"/LConn2 -- BusA/RConn2
  " 2"/LConn1 -- BusA/RConn1
  BusC/RConn1 -- Wind Type IV Detailed v2.1 - 1/LConn1
  BusC/RConn2 -- Wind Type IV Detailed v2.1 - 1/LConn2
  BusC/RConn3 -- Wind Type IV Detailed v2.1 - 1/LConn3
  Three-Phase Breaker 4/RConn3 -- BusA/LConn3
  Three-Phase Breaker 4/RConn2 -- BusA/LConn2
  BusA/LConn1 -- Three-Phase Breaker 4/RConn1
  "Three-Phase Breaker "/LConn1 -- BusC1/RConn1
  BusC1/RConn2 -- "Three-Phase Breaker "/LConn2
  "Three-Phase Breaker "/LConn3 -- BusC1/RConn3
  " 2"/RConn1 -- BusC2/LConn1
  " 2"/RConn2 -- BusC2/LConn2
  " 2"/RConn3 -- BusC2/LConn3
  BusC2/RConn1 -- Wind Type IV Detailed v2.1 - 2/LConn1
  BusC2/RConn2 -- Wind Type IV Detailed v2.1 - 2/LConn2
  BusC2/RConn3 -- Wind Type IV Detailed v2.1 - 2/LConn3
  Three-Phase Breaker 9/LConn2 -- BusC3/RConn2
  Three-Phase Breaker 9/LConn3 -- BusC3/RConn3
  2500 MVA X0/X1=2/LConn3 -- Vac kV2/RConn3
  2500 MVA X0/X1=2/LConn2 -- Vac kV2/RConn2
  Vac kV2/RConn1 -- 2500 MVA X0/X1=2/LConn1
  Ground1/LConn1 -- Vac kV2/LConn1
  5 km series11/RConn2 -- Wind Type IV Detailed v2.1 - 11/LConn2
  5 km series11/LConn2 -- Three-Phase Breaker 9/RConn2
  5 km series11/LConn1 -- Three-Phase Breaker 9/RConn1
  5 km series11/RConn3 -- Wind Type IV Detailed v2.1 - 11/LConn3
  5 km series11/RConn1 -- Wind Type IV Detailed v2.1 - 11/LConn1
  5 km series11/LConn3 -- Three-Phase Breaker 9/RConn3
  Three-Phase Breaker 10/LConn1 -- " 3"/RConn1
  Three-Phase Breaker 10/LConn2 -- " 3"/RConn2
  Three-Phase Breaker 10/LConn3 -- " 3"/RConn3
  Three-Phase Breaker 10/RConn2 -- Three-Phase Breaker 22/LConn2 -- BusC3/LConn2
  BusC3/LConn3 -- Three-Phase Breaker 10/RConn3 -- Three-Phase Breaker 22/LConn3
  Three-Phase Breaker 10/RConn1 -- Three-Phase Breaker 22/LConn1 -- BusC3/LConn1
  Three-Phase Breaker 11/RConn1 -- " 3"/LConn1
  Three-Phase Breaker 11/RConn2 -- " 3"/LConn2
  Three-Phase Breaker 11/RConn3 -- " 3"/LConn3
  Three-Phase Breaker 23/LConn3 -- BusC8/RConn3 -- Three-Phase Breaker 11/LConn3
  Three-Phase Breaker 12/LConn2 -- BusC4/RConn2
  Three-Phase Breaker 14/RConn2 -- " 4"/LConn2
  5 km series17/RConn1 -- Wind Type IV Detailed v2.1 - 14/LConn1
  Three-Phase Breaker 13/RConn3 -- Three-Phase Breaker 22/RConn3 -- BusC4/LConn3
  5 km series17/LConn3 -- Three-Phase Breaker 12/RConn3
  5 km series17/RConn2 -- Wind Type IV Detailed v2.1 - 14/LConn2
  Three-Phase Breaker 13/RConn2 -- Three-Phase Breaker 22/RConn2 -- BusC4/LConn2
  5 km series17/LConn2 -- Three-Phase Breaker 12/RConn2
  Three-Phase Breaker 13/RConn1 -- BusC4/LConn1 -- Three-Phase Breaker 22/RConn1
  Three-Phase Breaker 13/LConn2 -- " 4"/RConn2
  Three-Phase Breaker 14/RConn3 -- " 4"/LConn3
  Three-Phase Breaker 13/LConn3 -- " 4"/RConn3
  Three-Phase Breaker 14/RConn1 -- " 4"/LConn1
  5 km series17/RConn3 -- Wind Type IV Detailed v2.1 - 14/LConn3
  Three-Phase Breaker 13/LConn1 -- " 4"/RConn1
  5 km series17/LConn1 -- Three-Phase Breaker 12/RConn1
  Three-Phase Breaker 23/RConn1 -- BusC9/LConn1 -- Three-Phase Breaker 14/LConn1
  Three-Phase Breaker 23/RConn2 -- BusC9/LConn2 -- Three-Phase Breaker 14/LConn2
  Three-Phase Breaker 23/RConn3 -- BusC9/LConn3 -- Three-Phase Breaker 14/LConn3
  BusC6/RConn3 -- Three-Phase Breaker 27/LConn3
  Three-Phase Breaker 27/LConn1 -- BusC6/RConn1
  Three-Phase Breaker 27/LConn2 -- BusC6/RConn2
  Three-Phase Breaker 39/LConn3 -- BusC10/RConn3 -- Three-Phase Breaker 26/LConn3
  BusC5/RConn2 -- Three-Phase Breaker 41/LConn2
  BusC6/LConn3 -- Three-Phase Breaker 28/RConn3 -- Three-Phase Breaker 38/RConn3
  BusC5/LConn2 -- Three-Phase Breaker 25/RConn2 -- Three-Phase Breaker 38/LConn2
  Three-Phase Breaker 28/RConn1 -- BusC6/LConn1 -- Three-Phase Breaker 38/RConn1
  Three-Phase Breaker 41/LConn3 -- BusC5/RConn3
  Three-Phase Breaker 39/LConn2 -- BusC10/RConn2 -- Three-Phase Breaker 26/LConn2
  Three-Phase Breaker 28/RConn2 -- Three-Phase Breaker 38/RConn2 -- BusC6/LConn2
  BusC5/LConn3 -- Three-Phase Breaker 25/RConn3 -- Three-Phase Breaker 38/LConn3
  BusC5/LConn1 -- Three-Phase Breaker 25/RConn1 -- Three-Phase Breaker 38/LConn1
  Three-Phase Breaker 39/LConn1 -- Three-Phase Breaker 26/LConn1 -- BusC10/RConn1
  5 km series28/LConn2 -- Three-Phase Breaker 27/RConn2
  Three-Phase Breaker 26/RConn2 -- " 5"/LConn2
  Three-Phase Breaker 39/RConn2 -- BusC11/LConn2 -- Three-Phase Breaker 29/LConn2
  Three-Phase Breaker 29/RConn1 -- " 6"/LConn1
  5 km series28/RConn3 -- Wind Type IV Detailed v2.1 - 24/LConn3
  Three-Phase Breaker 28/LConn1 -- " 6"/RConn1
  Three-Phase Breaker 28/LConn3 -- " 6"/RConn3
  Three-Phase Breaker 28/LConn2 -- " 6"/RConn2
  Three-Phase Breaker 39/RConn1 -- BusC11/LConn1 -- Three-Phase Breaker 29/LConn1
  5 km series28/RConn1 -- Wind Type IV Detailed v2.1 - 24/LConn1
  5 km series28/RConn2 -- Wind Type IV Detailed v2.1 - 24/LConn2
  Three-Phase Breaker 39/RConn3 -- Three-Phase Breaker 29/LConn3 -- BusC11/LConn3
  Three-Phase Breaker 29/RConn2 -- " 6"/LConn2
  5 km series34/RConn2 -- Wind Type IV Detailed v2.1 - 33/LConn2
  5 km series34/RConn1 -- Wind Type IV Detailed v2.1 - 33/LConn1
  5 km series28/LConn1 -- Three-Phase Breaker 27/RConn1
  Three-Phase Breaker 25/LConn2 -- " 5"/RConn2
  Three-Phase Breaker 29/RConn3 -- " 6"/LConn3
  5 km series34/RConn3 -- Wind Type IV Detailed v2.1 - 33/LConn3
  5 km series34/LConn1 -- Three-Phase Breaker 41/RConn1
  5 km series28/LConn3 -- Three-Phase Breaker 27/RConn3
  Three-Phase Breaker 26/RConn3 -- " 5"/LConn3
  Three-Phase Breaker 26/RConn1 -- " 5"/LConn1
  Three-Phase Breaker 25/LConn3 -- " 5"/RConn3
  5 km series34/LConn3 -- Three-Phase Breaker 41/RConn3
  Three-Phase Breaker 25/LConn1 -- " 5"/RConn1
  5 km series34/LConn2 -- Three-Phase Breaker 41/RConn2
  Three-Phase Breaker 23/LConn2 -- BusC8/RConn2 -- Three-Phase Breaker 11/LConn2
  Three-Phase Breaker 23/LConn1 -- BusC8/RConn1 -- Three-Phase Breaker 11/LConn1
  BusC9/RConn3 -- Three-Phase Breaker 3/RConn3
  Three-Phase Breaker 8/RConn1 -- BusC11/RConn1
  Three-Phase Breaker 9/LConn1 -- BusC3/RConn1
  Three-Phase Breaker 12/LConn1 -- BusC4/RConn1
  BusC4/RConn3 -- Three-Phase Breaker 12/LConn3
  Three-Phase Breaker 41/LConn1 -- BusC5/RConn1
  Three-Phase Breaker 6/RConn2 -- BusC10/LConn2
  BusC11/RConn3 -- Three-Phase Breaker 8/RConn3
  Three-Phase Breaker 3/RConn2 -- BusC9/RConn2
  Three-Phase Breaker 3/RConn1 -- BusC9/RConn1
  BusC10/LConn3 -- Three-Phase Breaker 6/RConn3
  BusC11/RConn2 -- Three-Phase Breaker 8/RConn2
  BusC10/LConn1 -- Three-Phase Breaker 6/RConn1
